simulink model "ElevatorPlant_Storage_A"  (R2015b)
(part 4 of 8)

        (junction 68772) -> (junction 68786) [order 2]
        (junction 68773) -> (junction 68779) [order 2]
        (junction 68774) -> (junction 68775) [order 2]
        (junction 68776) -> (junction 68775)
        (junction 68775) -> (junction 68777)
        (junction 68777) -> OpCl_doors.Button_detection.Max_Min_assignment.MIN [order 1] : [MIN_BUT>BUT_TEMP && not(UPDATE)]
        OpCl_doors.Button_detection.Max_Min_assignment.MIN -> (junction 68778)
        (junction 68777) -> (junction 68780) [order 2]
        (junction 68778) -> (junction 68781)
        (junction 68780) -> (junction 68779)
        (junction 68781) -> (junction 68780)
        (junction 68779) -> (junction 68782)
        (junction 68782) -> OpCl_doors.Button_detection.Max_Min_assignment.Updating_button_0 [order 1] : [MOTION==0]
        OpCl_doors.Button_detection.Max_Min_assignment.Updating_button_0 -> (junction 68783)
        (junction 68782) -> (junction 68784) [order 2]
        (junction 68783) -> (junction 68785)
        (junction 68784) -> OpCl_doors.Button_detection.Max_Min_assignment.Updating_button_1 [order 1] : [MOTION==1]
        OpCl_doors.Button_detection.Max_Min_assignment.Updating_button_1 -> (junction 68785)
        (junction 68784) -> (junction 68787) [order 2]
        (junction 68785) -> (junction 68788)
        (junction 68787) -> (junction 68786)
        (junction 68788) -> (junction 68787)
      state GoTo_PositionControl
        en:
        BUTTON=BUT_TEMP;
        FLAG=2;
      state Emergency
        en:
        FLAG_EMG=true;
        FLAG=4;
      state Timer_EME
        state Set_tmr
          en:
          Q_EME=true;
        state Counting
          en:
          ET_EME= ET_EME + 1;
          Q_EME=false;
        state Set
          en:
          IN_EME=true;
          PT_EME=3;
        (junction 68878) -> OpCl_doors.Button_detection.Timer_EME.Set_tmr [order 1] : [ET_EME==PT_EME]
        OpCl_doors.Button_detection.Timer_EME.Set_tmr -> (junction 68879)
        OpCl_doors.Button_detection.Timer_EME.Counting -> (junction 68878)
        (junction 68878) -> (junction 68879) [order 2]
        (default) -> OpCl_doors.Button_detection.Timer_EME.Set
        OpCl_doors.Button_detection.Timer_EME.Set -> (junction 68880)
        (junction 68880) -> OpCl_doors.Button_detection.Timer_EME.Counting [order 1] : [ET_EME<PT_EME]
        (junction 68880) -> (junction 68879) [order 2]
      state Not_Emergency
        en:
        IN_EME=false;
        ET_EME=0;
      state SwitchingOFF_LEDs
        en:
        LPD3=false;
        LPD2=false;
        LPS2=false;
        LPD1=false;
        LPS1=false;
        LPS0=false;
      (default) -> (junction 68479)
      (junction 68479) -> (junction 68480) [order 1] : [FLAG==1 && not(PUSHED)]
          | {BUTTON=FLOOR;
          | BUT_TEMP=BUTTON;
          | BUT_1=FLOOR;}
      (junction 68480) -> OpCl_doors.Button_detection.Timer_LL [order 1] : [not(FLAG_STOP)]
      OpCl_doors.Button_detection.Save_energy -> (junction 68481)
      OpCl_doors.Button_detection.Timer_LL -> OpCl_doors.Button_detection.Save_energy
      (junction 68480) -> (junction 68483) [order 2]
      (junction 68479) -> (junction 68482) [order 2]
      (junction 68481) -> (junction 68484)
      (junction 68483) -> (junction 68482)
      (junction 68484) -> (junction 68483)
      (junction 68482) -> OpCl_doors.Button_detection.BUTTON_CAR
      OpCl_doors.Button_detection.BUTTON_UP -> OpCl_doors.Button_detection.BUTTON_DOWN
      OpCl_doors.Button_detection.BUTTON_DOWN -> OpCl_doors.Button_detection.Max_Min_assignment
      OpCl_doors.Button_detection.Max_Min_assignment -> (junction 68485)
      OpCl_doors.Button_detection.BUTTON_CAR -> OpCl_doors.Button_detection.BUTTON_UP
      (junction 68485) -> (junction 68487)
      (junction 68487) -> (junction 68486)
      (junction 68486) -> (junction 68489)
      OpCl_doors.Button_detection.GoTo_PositionControl -> (junction 68488)
      (junction 68489) -> (junction 68490) [order 1] : [FLAG==1]
      (junction 68490) -> OpCl_doors.Button_detection.GoTo_PositionControl [order 1] : [PUSHED]
      (junction 68488) -> (junction 68492)
      (junction 68489) -> (junction 68500) [order 2]
      (junction 68490) -> (junction 68491) [order 2]
      (junction 68492) -> (junction 68491)
      (junction 68491) -> (junction 68494)
      OpCl_doors.Button_detection.Emergency -> (junction 68493)
      (junction 68494) -> OpCl_doors.Button_detection.Timer_EME [order 1] : [STOP]
          | {IN_LL=false; ET_LL=0;FLAG=1;}
      OpCl_doors.Button_detection.Timer_EME -> (junction 68495)
      (junction 68495) -> OpCl_doors.Button_detection.Emergency [order 1] : [Q_EME]
      (junction 68493) -> (junction 68497)
      (junction 68494) -> OpCl_doors.Button_detection.Not_Emergency [order 2]
      (junction 68495) -> (junction 68496) [order 2]
      (junction 68497) -> (junction 68496)
      (junction 68496) -> (junction 68499)
      OpCl_doors.Button_detection.Not_Emergency -> (junction 68499)
      OpCl_doors.Button_detection.SwitchingOFF_LEDs -> (junction 68498)
      (junction 68499) -> OpCl_doors.Button_detection.SwitchingOFF_LEDs [order 1] : [FLAG_STOP && FLAG==2]
      (junction 68498) -> (junction 68502)
      (junction 68499) -> (junction 68501) [order 2]
      (junction 68501) -> (junction 68500)
      (junction 68502) -> (junction 68501)
    state OpCl_1
      state Closing1
        state Reset
          state Reset_0
            en:
            LPS0=false;
            BUTTON_CAR(1)=false;
            BUTTON_UP(1)=false;
          state Reset_1
            en:
            LPS1=false;
            LPD1=false;
            BUTTON_CAR(2)=false;
            BUTTON_UP(2)=false;
            BUTTON_DOWN(2)=false;
          state Reset_2
            en:
            LPS2=false;
            LPD2=false;
            BUTTON_CAR(3)=false;
            BUTTON_UP(3)=false;
            BUTTON_DOWN(3)=false;
          state Reset_3
            en:
            LPD3=false;
            BUTTON_CAR(4)=false;
            BUTTON_DOWN(4)=false;
          (default) -> (junction 69446)
          (junction 69446) -> OpCl_doors.OpCl_1.Closing1.Reset.Reset_0 [order 1] : [FLOOR==0]
          OpCl_doors.OpCl_1.Closing1.Reset.Reset_0 -> (junction 69447)
          (junction 69446) -> (junction 69448) [order 2]
          (junction 69447) -> (junction 69449)
          (junction 69448) -> OpCl_doors.OpCl_1.Closing1.Reset.Reset_1 [order 1] : [FLOOR==1]
          OpCl_doors.OpCl_1.Closing1.Reset.Reset_1 -> (junction 69449)
          (junction 69448) -> (junction 69450) [order 2]
          (junction 69449) -> (junction 69451)
          (junction 69450) -> OpCl_doors.OpCl_1.Closing1.Reset.Reset_2 [order 1] : [FLOOR==2]
          OpCl_doors.OpCl_1.Closing1.Reset.Reset_2 -> (junction 69451)
          (junction 69450) -> (junction 69452) [order 2]
          (junction 69451) -> (junction 69453)
          (junction 69452) -> OpCl_doors.OpCl_1.Closing1.Reset.Reset_3 [order 1] : [FLOOR==3]
          OpCl_doors.OpCl_1.Closing1.Reset.Reset_3 -> (junction 69453)
          (junction 69452) -> (junction 69454) [order 2]
          (junction 69453) -> (junction 69455)
          (junction 69455) -> (junction 69454)
        state Timer_close
          state Set_tmr
            en: Q_cl=true;
          state Set
            en:PT_cl=5;
            IN_cl=true;
          state Counting
            en:ET_cl = ET_cl + 1;
            Q_cl=false;
          (junction 69479) -> OpCl_doors.OpCl_1.Closing1.Timer_close.Set_tmr [order 1] : [ET_cl==PT_cl]
          OpCl_doors.OpCl_1.Closing1.Timer_close.Set_tmr -> (junction 69480)
          (default) -> OpCl_doors.OpCl_1.Closing1.Timer_close.Set
          OpCl_doors.OpCl_1.Closing1.Timer_close.Counting -> (junction 69479)
          (junction 69479) -> (junction 69480) [order 2]
          OpCl_doors.OpCl_1.Closing1.Timer_close.Set -> (junction 69481)
          (junction 69481) -> OpCl_doors.OpCl_1.Closing1.Timer_close.Counting [order 1] : [ET_cl<PT_cl]
          (junction 69481) -> (junction 69480) [order 2]
        state Closing
          en: CP1=Q_cl;
        state Button_detection
          state Save_energy
            en:
            LL=not(Q_LL);
          state Timer_LL
            state Set_tmr
              en:
              Q_LL=true;
            state Counting
              en:
              ET_LL= ET_LL + 1;
              Q_LL=false;
            state Set
              en:
              IN_LL=true;
              PT_LL=10;
            (junction 69563) -> OpCl_doors.OpCl_1.Closing1.Button_detection.Timer_LL.Set_tmr [order 1] : [ET_LL==PT_LL]
            OpCl_doors.OpCl_1.Closing1.Button_detection.Timer_LL.Set_tmr -> (junction 69564)
            OpCl_doors.OpCl_1.Closing1.Button_detection.Timer_LL.Counting -> (junction 69563)
            (junction 69563) -> (junction 69564) [order 2]
            (default) -> OpCl_doors.OpCl_1.Closing1.Button_detection.Timer_LL.Set
            OpCl_doors.OpCl_1.Closing1.Button_detection.Timer_LL.Set -> (junction 69565)
            (junction 69565) -> OpCl_doors.OpCl_1.Closing1.Button_detection.Timer_LL.Counting [order 1] : [ET_LL<PT_LL]
            (junction 69565) -> (junction 69564) [order 2]
          state BUTTON_DOWN
            state Button_DOWN_1
              en:
              BUTTON_DOWN(2)=true;
              BUT_TEMP=1;
              LPD1=true;
              PUSHED=true;
              UPDATE=false;
              IN_LL=false; ET_LL=0;
            state First_but_1
              en:
              BUT_1=BUT_TEMP;
              FIRST_BUT=false;
            state Button_DOWN_2
              en:
              BUTTON_DOWN(3)=true;
              BUT_TEMP=2;
              LPD2=true;
              PUSHED=true;
              UPDATE=false;
              IN_LL=false; ET_LL=0;
            state First_but_2
              en:
              BUT_1=BUT_TEMP;
              FIRST_BUT=false;
            state Button_DOWN_3
              en:
              BUTTON_DOWN(4)=true;
              BUT_TEMP=3;
              LPD3=true;
              PUSHED=true;
              UPDATE=false;
              IN_LL=false; ET_LL=0;
            state First_but_3
              en:
              BUT_1=BUT_TEMP;
              FIRST_BUT=false;
            (default) -> (junction 69578)
            (junction 69578) -> OpCl_doors.OpCl_1.Closing1.Button_detection.BUTTON_DOWN.Button_DOWN_1 [order 1] : [PD1]
            OpCl_doors.OpCl_1.Closing1.Button_detection.BUTTON_DOWN.Button_DOWN_1 -> (junction 69579)
            (junction 69579) -> OpCl_doors.OpCl_1.Closing1.Button_detection.BUTTON_DOWN.First_but_1 [order 1] : [FIRST_BUT && not(RPC1)]
            OpCl_doors.OpCl_1.Closing1.Button_detection.BUTTON_DOWN.First_but_1 -> (junction 69580)
            (junction 69578) -> (junction 69581) [order 2]
            (junction 69579) -> (junction 69582) [order 2]
            (junction 69580) -> (junction 69583)
            (junction 69582) -> (junction 69581)
            (junction 69583) -> (junction 69582)
            (junction 69581) -> (junction 69584)
            (junction 69584) -> OpCl_doors.OpCl_1.Closing1.Button_detection.BUTTON_DOWN.Button_DOWN_2 [order 1] : [PD2]
            OpCl_doors.OpCl_1.Closing1.Button_detection.BUTTON_DOWN.Button_DOWN_2 -> (junction 69585)
            (junction 69585) -> OpCl_doors.OpCl_1.Closing1.Button_detection.BUTTON_DOWN.First_but_2 [order 1] : [FIRST_BUT && not(RPC2)]
            OpCl_doors.OpCl_1.Closing1.Button_detection.BUTTON_DOWN.First_but_2 -> (junction 69586)
            (junction 69584) -> (junction 69587) [order 2]
            (junction 69585) -> (junction 69588) [order 2]
            (junction 69586) -> (junction 69589)
            (junction 69588) -> (junction 69587)
            (junction 69589) -> (junction 69588)
            (junction 69587) -> (junction 69590)
            (junction 69590) -> OpCl_doors.OpCl_1.Closing1.Button_detection.BUTTON_DOWN.Button_DOWN_3 [order 1] : [PD3]
            OpCl_doors.OpCl_1.Closing1.Button_detection.BUTTON_DOWN.Button_DOWN_3 -> (junction 69591)
            (junction 69591) -> OpCl_doors.OpCl_1.Closing1.Button_detection.BUTTON_DOWN.First_but_3 [order 1] : [FIRST_BUT && not(RPC3)]
            OpCl_doors.OpCl_1.Closing1.Button_detection.BUTTON_DOWN.First_but_3 -> (junction 69592)
            (junction 69590) -> (junction 69593) [order 2]
            (junction 69591) -> (junction 69594) [order 2]
            (junction 69592) -> (junction 69595)
            (junction 69594) -> (junction 69593)
            (junction 69595) -> (junction 69594)
          state BUTTON_CAR
            state Button_CAR_0
              en:
              BUTTON_CAR(1)=true;
              BUT_TEMP=0;
              LPC0=true;
              PUSHED=true;
              UPDATE=false;
              IN_LL=false; ET_LL=0;
            state First_but_0
              en:
              BUT_1=BUT_TEMP;
              FIRST_BUT=false;
            state Button_CAR_1
              en:
              BUTTON_CAR(2)=true;
              BUT_TEMP=1;
              LPC1=true;
              PUSHED=true;
              UPDATE=false;
              IN_LL=false; ET_LL=0;
            state First_but_1
              en:
              BUT_1=BUT_TEMP;
              FIRST_BUT=false;
            state Button_CAR_2
              en:
              BUTTON_CAR(3)=true;
              BUT_TEMP=2;
              LPC2=true;
              PUSHED=true;
              UPDATE=false;
              IN_LL=false; ET_LL=0;
            state First_but_2
              en:
              BUT_1=BUT_TEMP;
              FIRST_BUT=false;
            state Button_CAR_3
              en:
              BUTTON_CAR(4)=true;
              BUT_TEMP=3;
              LPC3=true;
              PUSHED=true;
              UPDATE=false;
              IN_LL=false; ET_LL=0;
            state First_but_3
              en:
              BUT_1=BUT_TEMP;
              FIRST_BUT=false;
            (default) -> (junction 69633)
            (junction 69633) -> OpCl_doors.OpCl_1.Closing1.Button_detection.BUTTON_CAR.Button_CAR_0 [order 1] : [P0]
            OpCl_doors.OpCl_1.Closing1.Button_detection.BUTTON_CAR.Button_CAR_0 -> (junction 69634)
            (junction 69634) -> OpCl_doors.OpCl_1.Closing1.Button_detection.BUTTON_CAR.First_but_0 [order 1] : [FIRST_BUT && not(RPC0)]
            OpCl_doors.OpCl_1.Closing1.Button_detection.BUTTON_CAR.First_but_0 -> (junction 69635)
            (junction 69633) -> (junction 69636) [order 2]
            (junction 69634) -> (junction 69637) [order 2]
            (junction 69635) -> (junction 69638)
            (junction 69637) -> (junction 69636)
            (junction 69638) -> (junction 69637)
            (junction 69636) -> (junction 69641)
            OpCl_doors.OpCl_1.Closing1.Button_detection.BUTTON_CAR.Button_CAR_1 -> (junction 69639)
            (junction 69639) -> OpCl_doors.OpCl_1.Closing1.Button_detection.BUTTON_CAR.First_but_1 [order 1] : [FIRST_BUT && not(RPC1)]
            OpCl_doors.OpCl_1.Closing1.Button_detection.BUTTON_CAR.First_but_1 -> (junction 69640)
            (junction 69639) -> (junction 69643) [order 2]
            (junction 69640) -> (junction 69644)
            (junction 69641) -> OpCl_doors.OpCl_1.Closing1.Button_detection.BUTTON_CAR.Button_CAR_1 [order 1] : [P1]
            (junction 69641) -> (junction 69642) [order 2]
            (junction 69643) -> (junction 69642)
            (junction 69644) -> (junction 69643)
            (junction 69642) -> (junction 69645)
            (junction 69645) -> OpCl_doors.OpCl_1.Closing1.Button_detection.BUTTON_CAR.Button_CAR_2 [order 1] : [P2]
            OpCl_doors.OpCl_1.Closing1.Button_detection.BUTTON_CAR.Button_CAR_2 -> (junction 69646)
            (junction 69646) -> OpCl_doors.OpCl_1.Closing1.Button_detection.BUTTON_CAR.First_but_2 [order 1] : [FIRST_BUT && not(RPC2)]
            OpCl_doors.OpCl_1.Closing1.Button_detection.BUTTON_CAR.First_but_2 -> (junction 69647)
            (junction 69645) -> (junction 69648) [order 2]
            (junction 69646) -> (junction 69649) [order 2]
            (junction 69647) -> (junction 69650)
            (junction 69649) -> (junction 69648)
            (junction 69650) -> (junction 69649)
            (junction 69648) -> (junction 69651)
            (junction 69651) -> OpCl_doors.OpCl_1.Closing1.Button_detection.BUTTON_CAR.Button_CAR_3 [order 1] : [P3]
            OpCl_doors.OpCl_1.Closing1.Button_detection.BUTTON_CAR.Button_CAR_3 -> (junction 69652)
            (junction 69652) -> OpCl_doors.OpCl_1.Closing1.Button_detection.BUTTON_CAR.First_but_3 [order 1] : [FIRST_BUT && not(RPC3)]
            OpCl_doors.OpCl_1.Closing1.Button_detection.BUTTON_CAR.First_but_3 -> (junction 69653)
            (junction 69651) -> (junction 69654) [order 2]
            (junction 69652) -> (junction 69655) [order 2]
            (junction 69653) -> (junction 69656)
            (junction 69655) -> (junction 69654)
            (junction 69656) -> (junction 69655)
          state BUTTON_UP
            state Button_UP_0
              en:
              BUTTON_UP(1)=true;
              BUT_TEMP=0;
              LPS0=true;
              PUSHED=true;
              UPDATE=false;
              IN_LL=false; ET_LL=0;
            state First_but_0
              en:
              BUT_1=BUT_TEMP;
              FIRST_BUT=false;
            state Button_UP_1
              en:
              BUTTON_UP(2)=true;
              BUT_TEMP=1;
              LPS1=true;
              PUSHED=true;
              UPDATE=false;
              IN_LL=false; ET_LL=0;
            state First_but_1
              en:
              BUT_1=BUT_TEMP;
              FIRST_BUT=false;
            state Button_UP_2
              en:
              BUTTON_UP(3)=true;
              BUT_TEMP=2;
              LPS2=true;
              PUSHED=true;
              UPDATE=false;
              IN_LL=false; ET_LL=0;
            state First_but_2
              en:
              BUT_1=BUT_TEMP;
              FIRST_BUT=false;
            (junction 69706) -> OpCl_doors.OpCl_1.Closing1.Button_detection.BUTTON_UP.Button_UP_0 [order 1] : [PS0]
            OpCl_doors.OpCl_1.Closing1.Button_detection.BUTTON_UP.Button_UP_0 -> (junction 69707)
            (junction 69707) -> OpCl_doors.OpCl_1.Closing1.Button_detection.BUTTON_UP.First_but_0 [order 1] : [FIRST_BUT && not(RPC0)]
            OpCl_doors.OpCl_1.Closing1.Button_detection.BUTTON_UP.First_but_0 -> (junction 69708)
            (default) -> (junction 69706)
            (junction 69706) -> (junction 69711) [order 2]
            (junction 69707) -> (junction 69709) [order 2]
            (junction 69708) -> (junction 69710)
            (junction 69710) -> (junction 69709)
            (junction 69709) -> (junction 69711)
            (junction 69711) -> (junction 69712)
            (junction 69712) -> OpCl_doors.OpCl_1.Closing1.Button_detection.BUTTON_UP.Button_UP_1 [order 1] : [PS1]
            OpCl_doors.OpCl_1.Closing1.Button_detection.BUTTON_UP.Button_UP_1 -> (junction 69713)
            (junction 69713) -> OpCl_doors.OpCl_1.Closing1.Button_detection.BUTTON_UP.First_but_1 [order 1] : [FIRST_BUT && not(RPC1)]
            OpCl_doors.OpCl_1.Closing1.Button_detection.BUTTON_UP.First_but_1 -> (junction 69714)
            (junction 69712) -> (junction 69715) [order 2]
            (junction 69713) -> (junction 69716) [order 2]
            (junction 69714) -> (junction 69717)
            (junction 69716) -> (junction 69715)
            (junction 69717) -> (junction 69716)
            (junction 69715) -> (junction 69719)
            OpCl_doors.OpCl_1.Closing1.Button_detection.BUTTON_UP.First_but_2 -> (junction 69718)
            (junction 69718) -> (junction 69723)
            (junction 69719) -> OpCl_doors.OpCl_1.Closing1.Button_detection.BUTTON_UP.Button_UP_2 [order 1] : [PS2]
            OpCl_doors.OpCl_1.Closing1.Button_detection.BUTTON_UP.Button_UP_2 -> (junction 69720)
            (junction 69720) -> OpCl_doors.OpCl_1.Closing1.Button_detection.BUTTON_UP.First_but_2 [order 1] : [FIRST_BUT && not(RPC2)]
            (junction 69719) -> (junction 69721) [order 2]
            (junction 69720) -> (junction 69722) [order 2]
            (junction 69722) -> (junction 69721)
            (junction 69723) -> (junction 69722)
          state Max_Min_assignment
            state Min_but
              en:
              BUTTON=MIN_BUT;
            state Max_but
              en:
              BUTTON=MAX_BUT;
            state First_but
              en:
              BUTTON=BUT_1;
            state Max_but1
              en:
              MAX_BUT=2;
            state Max_but2
              en:
              MAX_BUT=1;
            state Max_but3
              en:
              MAX_BUT=0;
            state Min_but1
              en:
              MIN_BUT=1;
            state Min_but2
              en:
              MIN_BUT=2;
            state Min_but3
              en:
              MIN_BUT=3;
            state MAX
              en:
              MAX_BUT=BUT_TEMP;
            state MIN
              en:
              MIN_BUT=BUT_TEMP;
            state Updating_button_0
              en:
              BUTTON=MAX_BUT;
            state Updating_button_1
              en:
              BUTTON=MIN_BUT;
            (junction 69761) -> OpCl_doors.OpCl_1.Closing1.Button_detection.Max_Min_assignment.Min_but [order 1] : [(MAX_BUT-FLOOR)>(FLOOR-MIN_BUT)]
            OpCl_doors.OpCl_1.Closing1.Button_detection.Max_Min_assignment.Min_but -> (junction 69762)
            (junction 69763) -> (junction 69761) [order 1] : [not(FLAG_STOP) && MOTION==2 && FLAG==3]
            (default) -> (junction 69763)
            (junction 69761) -> (junction 69764) [order 2]
            (junction 69762) -> (junction 69765)
            (junction 69763) -> (junction 69766) [order 2]
            (junction 69764) -> OpCl_doors.OpCl_1.Closing1.Button_detection.Max_Min_assignment.Max_but [order 1] : [(MAX_BUT-FLOOR)<(FLOOR-MIN_BUT)]
            OpCl_doors.OpCl_1.Closing1.Button_detection.Max_Min_assignment.Max_but -> (junction 69765)
            (junction 69764) -> OpCl_doors.OpCl_1.Closing1.Button_detection.Max_Min_assignment.First_but [order 2]
            (junction 69765) -> (junction 69768)
            OpCl_doors.OpCl_1.Closing1.Button_detection.Max_Min_assignment.First_but -> (junction 69767)
            (junction 69767) -> (junction 69766)
            (junction 69768) -> (junction 69767)
            (junction 69766) -> (junction 69769)
            (junction 69770) -> (junction 69771) [order 1] : [MOTION==0]
                | {MOTION=1;
                | UPDATE=true;}
            (junction 69771) -> OpCl_doors.OpCl_1.Closing1.Button_detection.Max_Min_assignment.Max_but1 [order 1] : [BUTTON_UP(2)]
            OpCl_doors.OpCl_1.Closing1.Button_detection.Max_Min_assignment.Max_but1 -> (junction 69772)
            (junction 69769) -> (junction 69770) [order 1] : [BUTTON==FLOOR && EXTEND]
                | {EXTEND=false;}
            (junction 69769) -> (junction 69783) [order 2]
            (junction 69770) -> (junction 69775) [order 2]
            (junction 69771) -> (junction 69773) [order 2]
            (junction 69772) -> (junction 69774)
            (junction 69773) -> OpCl_doors.OpCl_1.Closing1.Button_detection.Max_Min_assignment.Max_but2 [order 1] : [BUTTON_UP(1)]
            OpCl_doors.OpCl_1.Closing1.Button_detection.Max_Min_assignment.Max_but2 -> (junction 69774)
            (junction 69773) -> OpCl_doors.OpCl_1.Closing1.Button_detection.Max_Min_assignment.Max_but3 [order 2]
            (junction 69774) -> (junction 69777)
            OpCl_doors.OpCl_1.Closing1.Button_detection.Max_Min_assignment.Max_but3 -> (junction 69776)
            (junction 69776) -> (junction 69775)
            (junction 69777) -> (junction 69776)
            (junction 69775) -> (junction 69778)
            (junction 69778) -> (junction 69779) [order 1] : [MOTION==1]
                | {MOTION=0;
                | UPDATE=true;}
            (junction 69779) -> OpCl_doors.OpCl_1.Closing1.Button_detection.Max_Min_assignment.Min_but1 [order 1] : [BUTTON_DOWN(1)]
            OpCl_doors.OpCl_1.Closing1.Button_detection.Max_Min_assignment.Min_but1 -> (junction 69780)
            (junction 69778) -> (junction 69784) [order 2]
            (junction 69779) -> (junction 69781) [order 2]
            (junction 69780) -> (junction 69782)
            (junction 69781) -> OpCl_doors.OpCl_1.Closing1.Button_detection.Max_Min_assignment.Min_but2 [order 1] : [BUTTON_DOWN(2)]
            OpCl_doors.OpCl_1.Closing1.Button_detection.Max_Min_assignment.Min_but2 -> (junction 69782)
            (junction 69781) -> OpCl_doors.OpCl_1.Closing1.Button_detection.Max_Min_assignment.Min_but3 [order 2]
            (junction 69782) -> (junction 69786)
            OpCl_doors.OpCl_1.Closing1.Button_detection.Max_Min_assignment.Min_but3 -> (junction 69785)
            (junction 69784) -> (junction 69783)
            (junction 69785) -> (junction 69784)
            (junction 69786) -> (junction 69785)
            (junction 69783) -> (junction 69788)
            OpCl_doors.OpCl_1.Closing1.Button_detection.Max_Min_assignment.MAX -> (junction 69787)
            (junction 69788) -> (junction 69789) [order 1] : [PUSHED]
            (junction 69789) -> (junction 69790) [order 1] : [not(BUT_TEMP==FLOOR) || not(MOTION==2)]
            (junction 69790) -> OpCl_doors.OpCl_1.Closing1.Button_detection.Max_Min_assignment.MAX [order 1] : [MAX_BUT<BUT_TEMP && not(UPDATE)]
            (junction 69787) -> (junction 69792)
            (junction 69788) -> (junction 69802) [order 2]
            (junction 69789) -> (junction 69795) [order 2]
            (junction 69790) -> (junction 69791) [order 2]
            (junction 69792) -> (junction 69791)
            (junction 69791) -> (junction 69793)
            (junction 69793) -> OpCl_doors.OpCl_1.Closing1.Button_detection.Max_Min_assignment.MIN [order 1] : [MIN_BUT>BUT_TEMP && not(UPDATE)]
            OpCl_doors.OpCl_1.Closing1.Button_detection.Max_Min_assignment.MIN -> (junction 69794)
            (junction 69793) -> (junction 69796) [order 2]
            (junction 69794) -> (junction 69797)
            (junction 69796) -> (junction 69795)
            (junction 69797) -> (junction 69796)
            (junction 69795) -> (junction 69798)
            (junction 69798) -> OpCl_doors.OpCl_1.Closing1.Button_detection.Max_Min_assignment.Updating_button_0 [order 1] : [MOTION==0]
            OpCl_doors.OpCl_1.Closing1.Button_detection.Max_Min_assignment.Updating_button_0 -> (junction 69799)
            (junction 69798) -> (junction 69800) [order 2]
            (junction 69799) -> (junction 69801)
            (junction 69800) -> OpCl_doors.OpCl_1.Closing1.Button_detection.Max_Min_assignment.Updating_button_1 [order 1] : [MOTION==1]
            OpCl_doors.OpCl_1.Closing1.Button_detection.Max_Min_assignment.Updating_button_1 -> (junction 69801)
            (junction 69800) -> (junction 69803) [order 2]
            (junction 69801) -> (junction 69804)
            (junction 69803) -> (junction 69802)
            (junction 69804) -> (junction 69803)
          state GoTo_PositionControl
            en:
            BUTTON=BUT_TEMP;
            FLAG=2;
          state Emergency
            en:
            FLAG_EMG=true;
            FLAG=4;
          state Timer_EME
            state Set_tmr
              en:
              Q_EME=true;
            state Counting
              en:
              ET_EME= ET_EME + 1;
              Q_EME=false;
            state Set
              en:
              IN_EME=true;
              PT_EME=3;
            (junction 69894) -> OpCl_doors.OpCl_1.Closing1.Button_detection.Timer_EME.Set_tmr [order 1] : [ET_EME==PT_EME]
            OpCl_doors.OpCl_1.Closing1.Button_detection.Timer_EME.Set_tmr -> (junction 69895)
            OpCl_doors.OpCl_1.Closing1.Button_detection.Timer_EME.Counting -> (junction 69894)
            (junction 69894) -> (junction 69895) [order 2]
            (default) -> OpCl_doors.OpCl_1.Closing1.Button_detection.Timer_EME.Set
            OpCl_doors.OpCl_1.Closing1.Button_detection.Timer_EME.Set -> (junction 69896)
            (junction 69896) -> OpCl_doors.OpCl_1.Closing1.Button_detection.Timer_EME.Counting [order 1] : [ET_EME<PT_EME]
            (junction 69896) -> (junction 69895) [order 2]
          state Not_Emergency
            en:
            IN_EME=false;
            ET_EME=0;
          state SwitchingOFF_LEDs
            en:
            LPD3=false;
            LPD2=false;
            LPS2=false;
            LPD1=false;
            LPS1=false;
            LPS0=false;
          (default) -> (junction 69495)
          (junction 69495) -> (junction 69496) [order 1] : [FLAG==1 && not(PUSHED)]
              | {BUTTON=FLOOR;
              | BUT_TEMP=BUTTON;
              | BUT_1=FLOOR;}
          (junction 69496) -> OpCl_doors.OpCl_1.Closing1.Button_detection.Timer_LL [order 1] : [not(FLAG_STOP)]
          OpCl_doors.OpCl_1.Closing1.Button_detection.Save_energy -> (junction 69497)
          OpCl_doors.OpCl_1.Closing1.Button_detection.Timer_LL -> OpCl_doors.OpCl_1.Closing1.Button_detection.Save_energy
          (junction 69496) -> (junction 69499) [order 2]
          (junction 69495) -> (junction 69498) [order 2]
          (junction 69497) -> (junction 69500)
          (junction 69499) -> (junction 69498)
          (junction 69500) -> (junction 69499)
          (junction 69498) -> OpCl_doors.OpCl_1.Closing1.Button_detection.BUTTON_CAR
          OpCl_doors.OpCl_1.Closing1.Button_detection.BUTTON_UP -> OpCl_doors.OpCl_1.Closing1.Button_detection.BUTTON_DOWN
          OpCl_doors.OpCl_1.Closing1.Button_detection.BUTTON_DOWN -> OpCl_doors.OpCl_1.Closing1.Button_detection.Max_Min_assignment
          OpCl_doors.OpCl_1.Closing1.Button_detection.Max_Min_assignment -> (junction 69501)
          OpCl_doors.OpCl_1.Closing1.Button_detection.BUTTON_CAR -> OpCl_doors.OpCl_1.Closing1.Button_detection.BUTTON_UP
          (junction 69501) -> (junction 69503)
          (junction 69503) -> (junction 69502)
          (junction 69502) -> (junction 69505)
          OpCl_doors.OpCl_1.Closing1.Button_detection.GoTo_PositionControl -> (junction 69504)
          (junction 69505) -> (junction 69506) [order 1] : [FLAG==1]
          (junction 69506) -> OpCl_doors.OpCl_1.Closing1.Button_detection.GoTo_PositionControl [order 1] : [PUSHED]
          (junction 69504) -> (junction 69508)
          (junction 69505) -> (junction 69516) [order 2]
          (junction 69506) -> (junction 69507) [order 2]
          (junction 69508) -> (junction 69507)
          (junction 69507) -> (junction 69510)
          OpCl_doors.OpCl_1.Closing1.Button_detection.Emergency -> (junction 69509)
          (junction 69510) -> OpCl_doors.OpCl_1.Closing1.Button_detection.Timer_EME [order 1] : [STOP]
              | {IN_LL=false; ET_LL=0;FLAG=1;}
          OpCl_doors.OpCl_1.Closing1.Button_detection.Timer_EME -> (junction 69511)
          (junction 69511) -> OpCl_doors.OpCl_1.Closing1.Button_detection.Emergency [order 1] : [Q_EME]
          (junction 69509) -> (junction 69513)
          (junction 69510) -> OpCl_doors.OpCl_1.Closing1.Button_detection.Not_Emergency [order 2]
          (junction 69511) -> (junction 69512) [order 2]
          (junction 69513) -> (junction 69512)
          (junction 69512) -> (junction 69515)
          OpCl_doors.OpCl_1.Closing1.Button_detection.Not_Emergency -> (junction 69515)
          OpCl_doors.OpCl_1.Closing1.Button_detection.SwitchingOFF_LEDs -> (junction 69514)
          (junction 69515) -> OpCl_doors.OpCl_1.Closing1.Button_detection.SwitchingOFF_LEDs [order 1] : [FLAG_STOP && FLAG==2]
          (junction 69514) -> (junction 69518)
          (junction 69515) -> (junction 69517) [order 2]
          (junction 69517) -> (junction 69516)
          (junction 69518) -> (junction 69517)
        state Extending
          en:
          EXTEND=true;
        state Stop_Closing
          en:
          CP1=false;
          FLAG_OD=false;
          OBS=false;
          ET_cl=0;
          IN_cl=false;
        state GoTo_PositionControl
          en: FLAG=2;
        state GoTo_BUttonDetection
          en:
          MOTION=2;
          MAX_BUT=0;
          MIN_BUT=3;
          PUSHED=false;
          FIRST_BUT=true;
          FLAG=1;
          UPDATE=false;
        state Closing1
          en:CP1=true;
        state Stop_Closing1
          en:CP1=false;
        OpCl_doors.OpCl_1.Closing1.Reset -> OpCl_doors.OpCl_1.Closing1.Timer_close
        (default) -> (junction 69406)
        (junction 69406) -> OpCl_doors.OpCl_1.Closing1.Reset [order 1] : [not(FLAG==0) && not(FLAG==4)]
        OpCl_doors.OpCl_1.Closing1.Timer_close -> (junction 69407)
        (junction 69407) -> OpCl_doors.OpCl_1.Closing1.Closing [order 1] : [not(PC1)]
        OpCl_doors.OpCl_1.Closing1.Button_detection -> (junction 69408)
        OpCl_doors.OpCl_1.Closing1.Closing -> OpCl_doors.OpCl_1.Closing1.Button_detection
        (junction 69406) -> (junction 69416) [order 2]
        (junction 69407) -> (junction 69409) [order 2]
        (junction 69408) -> (junction 69414)
        (junction 69409) -> OpCl_doors.OpCl_1.Closing1.Extending [order 1] : [BUTTON==FLOOR]
        (junction 69409) -> (junction 69411) [order 2]
        OpCl_doors.OpCl_1.Closing1.Extending -> (junction 69410)
        (junction 69410) -> (junction 69411)
        (junction 69411) -> OpCl_doors.OpCl_1.Closing1.Stop_Closing
        OpCl_doors.OpCl_1.Closing1.Stop_Closing -> (junction 69412)
        (junction 69412) -> OpCl_doors.OpCl_1.Closing1.GoTo_PositionControl [order 2]
        (junction 69412) -> OpCl_doors.OpCl_1.Closing1.GoTo_BUttonDetection [order 1] : [not(BUTTON_CAR(1) || BUTTON_CAR(2) || BUTTON_CAR(3) || BUTTON_CAR(4) || BUTTON_UP(1) || BUTTON_UP(2) || BUTTON_UP(3) || BUTTON_DOWN(2) || BUTTON_DOWN(3) || BUTTON_DOWN(4))]
        OpCl_doors.OpCl_1.Closing1.GoTo_PositionControl -> (junction 69413)
        OpCl_doors.OpCl_1.Closing1.GoTo_BUttonDetection -> (junction 69413)
        (junction 69413) -> (junction 69414)
        (junction 69414) -> (junction 69415)
        (junction 69415) -> (junction 69417)
        (junction 69416) -> OpCl_doors.OpCl_1.Closing1.Closing1 [order 1] : [not(PC1)]
        OpCl_doors.OpCl_1.Closing1.Closing1 -> (junction 69417)
        (junction 69416) -> OpCl_doors.OpCl_1.Closing1.Stop_Closing1 [order 2]
        OpCl_doors.OpCl_1.Closing1.Stop_Closing1 -> (junction 69417)
      state StopClosing
        en: CP1=false;
        FLAG_OD=false;
      state Opening1
        state Opening
          en:AP1=Q_op;
        state People_IN
          state Check_People_IN
            en:
            COUNTER_IN=false;
          state People_KID_IN
            en:
            WEIGHT=WEIGHT+30;
            KIDS=KIDS+1;
          state People_WOMAN_IN
            en:
            WEIGHT=WEIGHT+55;
            WOMEN=WOMEN+1;
          state People_MAN_IN
            en:
            WEIGHT=WEIGHT+75;
            MEN=MEN+1;
          state People_FATGUY_IN
            en:
            WEIGHT=WEIGHT+100;
            FATGUYS=FATGUYS+1;
          state Re_Ready_IN
            en:
            COUNTER_IN=true;
          (default) -> (junction 88272)
          (junction 88272) -> OpCl_doors.OpCl_1.Opening1.People_IN.Check_People_IN [order 1] : [COUNTER_IN]
          OpCl_doors.OpCl_1.Opening1.People_IN.Check_People_IN -> (junction 88273)
          (junction 88273) -> OpCl_doors.OpCl_1.Opening1.People_IN.People_KID_IN [order 1] : [KID_IN]
          OpCl_doors.OpCl_1.Opening1.People_IN.People_KID_IN -> (junction 88274)
          (junction 88272) -> (junction 88281) [order 2]
          (junction 88273) -> (junction 88275) [order 2]
          (junction 88274) -> (junction 88276)
          (junction 88275) -> OpCl_doors.OpCl_1.Opening1.People_IN.People_WOMAN_IN [order 1] : [WOMAN_IN]
          OpCl_doors.OpCl_1.Opening1.People_IN.People_WOMAN_IN -> (junction 88276)
          (junction 88275) -> (junction 88277) [order 2]
          (junction 88276) -> (junction 88278)
          (junction 88277) -> OpCl_doors.OpCl_1.Opening1.People_IN.People_MAN_IN [order 1] : [MAN_IN]
          OpCl_doors.OpCl_1.Opening1.People_IN.People_MAN_IN -> (junction 88278)
          (junction 88277) -> (junction 88279) [order 2]
          (junction 88278) -> (junction 88280)
          (junction 88279) -> OpCl_doors.OpCl_1.Opening1.People_IN.People_FATGUY_IN [order 1] : [FATGUY_IN]
          OpCl_doors.OpCl_1.Opening1.People_IN.People_FATGUY_IN -> (junction 88280)
          (junction 88279) -> (junction 88282) [order 2]
          (junction 88280) -> (junction 88283)
          (junction 88282) -> (junction 88281)
          (junction 88283) -> (junction 88282)
          (junction 88281) -> (junction 88284)
          (junction 88284) -> OpCl_doors.OpCl_1.Opening1.People_IN.Re_Ready_IN [order 1] : [not(KID_IN|| WOMAN_IN || MAN_IN || FATGUY_IN)]
          (junction 88284) -> (junction 88285) [order 2]
          OpCl_doors.OpCl_1.Opening1.People_IN.Re_Ready_IN -> (junction 88286)
          (junction 88286) -> (junction 88285)
        state Timer_open
          state Set_tmr
            en: Q_op=true;
          state Set
            en:PT_op=2;
            IN_op=true;
          state Counting
            en:ET_op = ET_op + 1;
            Q_op=false;
          (junction 88321) -> OpCl_doors.OpCl_1.Opening1.Timer_open.Set_tmr [order 1] : [ET_op==PT_op]
          OpCl_doors.OpCl_1.Opening1.Timer_open.Set_tmr -> (junction 88322)
          (default) -> OpCl_doors.OpCl_1.Opening1.Timer_open.Set
          OpCl_doors.OpCl_1.Opening1.Timer_open.Counting -> (junction 88321)
          (junction 88321) -> (junction 88322) [order 2]
          OpCl_doors.OpCl_1.Opening1.Timer_open.Set -> (junction 88323)
          (junction 88323) -> OpCl_doors.OpCl_1.Opening1.Timer_open.Counting [order 1] : [ET_op<PT_op]
          (junction 88323) -> (junction 88322) [order 2]
        state Stop_Opening
          en:AP1=false;
          FLAG_OD=true;
          OBS=true;
          IN_op=false;
          ET_op=0;
        state People_OUT
          state Check_People_OUT
            en:
            COUNTER_OUT=false;
          state People_KID_OUT
            en:
            WEIGHT=WEIGHT-30;
            KIDS=KIDS-1;
          state People_WOMAN_OUT
            en:
            WEIGHT=WEIGHT-55;
            WOMEN=WOMEN-1;
          state People_MAN_OUT
            en:
            WEIGHT=WEIGHT-75;
            MEN=MEN-1;
          state People_FATGUY_OUT
            en:
            WEIGHT=WEIGHT-100;
            FATGUYS=FATGUYS-1;
          state Re_Ready_OUT
            en:
            COUNTER_OUT=true;
          (default) -> (junction 88337)
          (junction 88337) -> OpCl_doors.OpCl_1.Opening1.People_OUT.Check_People_OUT [order 1] : [COUNTER_OUT]
          OpCl_doors.OpCl_1.Opening1.People_OUT.Check_People_OUT -> (junction 88338)
          (junction 88338) -> OpCl_doors.OpCl_1.Opening1.People_OUT.People_KID_OUT [order 1] : [KID_OUT && KIDS>0 ]
          OpCl_doors.OpCl_1.Opening1.People_OUT.People_KID_OUT -> (junction 88339)
          (junction 88337) -> (junction 88346) [order 2]
          (junction 88338) -> (junction 88340) [order 2]
          (junction 88339) -> (junction 88341)
          (junction 88340) -> OpCl_doors.OpCl_1.Opening1.People_OUT.People_WOMAN_OUT [order 1] : [WOMAN_OUT && WOMEN>0]
          OpCl_doors.OpCl_1.Opening1.People_OUT.People_WOMAN_OUT -> (junction 88341)
          (junction 88341) -> (junction 88343)
          (junction 88340) -> (junction 88342) [order 2]
          (junction 88342) -> OpCl_doors.OpCl_1.Opening1.People_OUT.People_MAN_OUT [order 1] : [MAN_OUT && MEN>0]
          OpCl_doors.OpCl_1.Opening1.People_OUT.People_MAN_OUT -> (junction 88343)
          (junction 88342) -> (junction 88344) [order 2]
          (junction 88343) -> (junction 88345)
          (junction 88344) -> OpCl_doors.OpCl_1.Opening1.People_OUT.People_FATGUY_OUT [order 1] : [FATGUY_OUT && FATGUYS>0]
          OpCl_doors.OpCl_1.Opening1.People_OUT.People_FATGUY_OUT -> (junction 88345)
          (junction 88344) -> (junction 88347) [order 2]
          (junction 88345) -> (junction 88348)
          (junction 88347) -> (junction 88346)
          (junction 88348) -> (junction 88347)
          (junction 88346) -> (junction 88349)
          (junction 88349) -> OpCl_doors.OpCl_1.Opening1.People_OUT.Re_Ready_OUT [order 1] : [not(KID_OUT || WOMAN_OUT || MAN_OUT || FATGUY_OUT)]
          (junction 88349) -> (junction 88350) [order 2]
          OpCl_doors.OpCl_1.Opening1.People_OUT.Re_Ready_OUT -> (junction 88351)
          (junction 88351) -> (junction 88350)
        state Button_detection
          state Save_energy
            en:
            LL=not(Q_LL);
          state Timer_LL
            state Set_tmr
              en:
              Q_LL=true;
            state Counting
              en:
              ET_LL= ET_LL + 1;
              Q_LL=false;
            state Set
              en:
              IN_LL=true;
              PT_LL=10;
            (junction 88454) -> OpCl_doors.OpCl_1.Opening1.Button_detection.Timer_LL.Set_tmr [order 1] : [ET_LL==PT_LL]
            OpCl_doors.OpCl_1.Opening1.Button_detection.Timer_LL.Set_tmr -> (junction 88455)
            OpCl_doors.OpCl_1.Opening1.Button_detection.Timer_LL.Counting -> (junction 88454)
            (junction 88454) -> (junction 88455) [order 2]
            (default) -> OpCl_doors.OpCl_1.Opening1.Button_detection.Timer_LL.Set
            OpCl_doors.OpCl_1.Opening1.Button_detection.Timer_LL.Set -> (junction 88456)
            (junction 88456) -> OpCl_doors.OpCl_1.Opening1.Button_detection.Timer_LL.Counting [order 1] : [ET_LL<PT_LL]
            (junction 88456) -> (junction 88455) [order 2]
          state BUTTON_DOWN
            state Button_DOWN_1
              en:
              BUTTON_DOWN(2)=true;
              BUT_TEMP=1;
              LPD1=true;
              PUSHED=true;
              UPDATE=false;
              IN_LL=false; ET_LL=0;
            state First_but_1
              en:
              BUT_1=BUT_TEMP;
              FIRST_BUT=false;
            state Button_DOWN_2
              en:
              BUTTON_DOWN(3)=true;
              BUT_TEMP=2;
              LPD2=true;
              PUSHED=true;
              UPDATE=false;
              IN_LL=false; ET_LL=0;
            state First_but_2
              en:
              BUT_1=BUT_TEMP;
              FIRST_BUT=false;
            state Button_DOWN_3
              en:
              BUTTON_DOWN(4)=true;
              BUT_TEMP=3;
              LPD3=true;
              PUSHED=true;
              UPDATE=false;
              IN_LL=false; ET_LL=0;
            state First_but_3
              en:
              BUT_1=BUT_TEMP;
              FIRST_BUT=false;
            (default) -> (junction 88469)
            (junction 88469) -> OpCl_doors.OpCl_1.Opening1.Button_detection.BUTTON_DOWN.Button_DOWN_1 [order 1] : [PD1]
            OpCl_doors.OpCl_1.Opening1.Button_detection.BUTTON_DOWN.Button_DOWN_1 -> (junction 88470)
            (junction 88470) -> OpCl_doors.OpCl_1.Opening1.Button_detection.BUTTON_DOWN.First_but_1 [order 1] : [FIRST_BUT && not(RPC1)]
            OpCl_doors.OpCl_1.Opening1.Button_detection.BUTTON_DOWN.First_but_1 -> (junction 88471)
            (junction 88469) -> (junction 88472) [order 2]
            (junction 88470) -> (junction 88473) [order 2]
            (junction 88471) -> (junction 88474)
            (junction 88473) -> (junction 88472)
            (junction 88474) -> (junction 88473)
            (junction 88472) -> (junction 88475)
            (junction 88475) -> OpCl_doors.OpCl_1.Opening1.Button_detection.BUTTON_DOWN.Button_DOWN_2 [order 1] : [PD2]
            OpCl_doors.OpCl_1.Opening1.Button_detection.BUTTON_DOWN.Button_DOWN_2 -> (junction 88476)
            (junction 88476) -> OpCl_doors.OpCl_1.Opening1.Button_detection.BUTTON_DOWN.First_but_2 [order 1] : [FIRST_BUT && not(RPC2)]
            OpCl_doors.OpCl_1.Opening1.Button_detection.BUTTON_DOWN.First_but_2 -> (junction 88477)
            (junction 88475) -> (junction 88478) [order 2]
            (junction 88476) -> (junction 88479) [order 2]
            (junction 88477) -> (junction 88480)
            (junction 88479) -> (junction 88478)
            (junction 88480) -> (junction 88479)
            (junction 88478) -> (junction 88481)
            (junction 88481) -> OpCl_doors.OpCl_1.Opening1.Button_detection.BUTTON_DOWN.Button_DOWN_3 [order 1] : [PD3]
            OpCl_doors.OpCl_1.Opening1.Button_detection.BUTTON_DOWN.Button_DOWN_3 -> (junction 88482)
            (junction 88482) -> OpCl_doors.OpCl_1.Opening1.Button_detection.BUTTON_DOWN.First_but_3 [order 1] : [FIRST_BUT && not(RPC3)]
            OpCl_doors.OpCl_1.Opening1.Button_detection.BUTTON_DOWN.First_but_3 -> (junction 88483)
            (junction 88481) -> (junction 88484) [order 2]
            (junction 88482) -> (junction 88485) [order 2]
            (junction 88483) -> (junction 88486)
            (junction 88485) -> (junction 88484)
            (junction 88486) -> (junction 88485)
          state BUTTON_CAR
            state Button_CAR_0
              en:
              BUTTON_CAR(1)=true;
              BUT_TEMP=0;
              LPC0=true;
              PUSHED=true;
              UPDATE=false;
              IN_LL=false; ET_LL=0;
            state First_but_0
              en:
              BUT_1=BUT_TEMP;
              FIRST_BUT=false;
            state Button_CAR_1
              en:
              BUTTON_CAR(2)=true;
              BUT_TEMP=1;
              LPC1=true;
              PUSHED=true;
              UPDATE=false;
              IN_LL=false; ET_LL=0;
            state First_but_1
              en:
              BUT_1=BUT_TEMP;
              FIRST_BUT=false;
            state Button_CAR_2
              en:
              BUTTON_CAR(3)=true;
              BUT_TEMP=2;
              LPC2=true;
              PUSHED=true;
              UPDATE=false;
              IN_LL=false; ET_LL=0;
            state First_but_2
              en:
              BUT_1=BUT_TEMP;
              FIRST_BUT=false;
            state Button_CAR_3
              en:
              BUTTON_CAR(4)=true;
              BUT_TEMP=3;
              LPC3=true;
              PUSHED=true;
              UPDATE=false;
              IN_LL=false; ET_LL=0;
            state First_but_3
              en:
              BUT_1=BUT_TEMP;
              FIRST_BUT=false;
            (default) -> (junction 88524)
            (junction 88524) -> OpCl_doors.OpCl_1.Opening1.Button_detection.BUTTON_CAR.Button_CAR_0 [order 1] : [P0]
            OpCl_doors.OpCl_1.Opening1.Button_detection.BUTTON_CAR.Button_CAR_0 -> (junction 88525)
            (junction 88525) -> OpCl_doors.OpCl_1.Opening1.Button_detection.BUTTON_CAR.First_but_0 [order 1] : [FIRST_BUT && not(RPC0)]
            OpCl_doors.OpCl_1.Opening1.Button_detection.BUTTON_CAR.First_but_0 -> (junction 88526)
            (junction 88524) -> (junction 88527) [order 2]
            (junction 88525) -> (junction 88528) [order 2]
            (junction 88526) -> (junction 88529)
            (junction 88528) -> (junction 88527)
            (junction 88529) -> (junction 88528)
            (junction 88527) -> (junction 88532)
            OpCl_doors.OpCl_1.Opening1.Button_detection.BUTTON_CAR.Button_CAR_1 -> (junction 88530)
            (junction 88530) -> OpCl_doors.OpCl_1.Opening1.Button_detection.BUTTON_CAR.First_but_1 [order 1] : [FIRST_BUT && not(RPC1)]
            OpCl_doors.OpCl_1.Opening1.Button_detection.BUTTON_CAR.First_but_1 -> (junction 88531)
            (junction 88530) -> (junction 88534) [order 2]
            (junction 88531) -> (junction 88535)
            (junction 88532) -> OpCl_doors.OpCl_1.Opening1.Button_detection.BUTTON_CAR.Button_CAR_1 [order 1] : [P1]
            (junction 88532) -> (junction 88533) [order 2]
            (junction 88534) -> (junction 88533)
            (junction 88535) -> (junction 88534)
            (junction 88533) -> (junction 88536)
            (junction 88536) -> OpCl_doors.OpCl_1.Opening1.Button_detection.BUTTON_CAR.Button_CAR_2 [order 1] : [P2]
            OpCl_doors.OpCl_1.Opening1.Button_detection.BUTTON_CAR.Button_CAR_2 -> (junction 88537)
            (junction 88537) -> OpCl_doors.OpCl_1.Opening1.Button_detection.BUTTON_CAR.First_but_2 [order 1] : [FIRST_BUT && not(RPC2)]
            OpCl_doors.OpCl_1.Opening1.Button_detection.BUTTON_CAR.First_but_2 -> (junction 88538)
            (junction 88536) -> (junction 88539) [order 2]
            (junction 88537) -> (junction 88540) [order 2]
            (junction 88538) -> (junction 88541)
            (junction 88540) -> (junction 88539)
            (junction 88541) -> (junction 88540)
            (junction 88539) -> (junction 88542)
            (junction 88542) -> OpCl_doors.OpCl_1.Opening1.Button_detection.BUTTON_CAR.Button_CAR_3 [order 1] : [P3]
            OpCl_doors.OpCl_1.Opening1.Button_detection.BUTTON_CAR.Button_CAR_3 -> (junction 88543)
            (junction 88543) -> OpCl_doors.OpCl_1.Opening1.Button_detection.BUTTON_CAR.First_but_3 [order 1] : [FIRST_BUT && not(RPC3)]
            OpCl_doors.OpCl_1.Opening1.Button_detection.BUTTON_CAR.First_but_3 -> (junction 88544)
            (junction 88542) -> (junction 88545) [order 2]
            (junction 88543) -> (junction 88546) [order 2]
            (junction 88544) -> (junction 88547)
            (junction 88546) -> (junction 88545)
            (junction 88547) -> (junction 88546)
          state BUTTON_UP
            state Button_UP_0
              en:
              BUTTON_UP(1)=true;
              BUT_TEMP=0;
              LPS0=true;
              PUSHED=true;
              UPDATE=false;
              IN_LL=false; ET_LL=0;
            state First_but_0
              en:
              BUT_1=BUT_TEMP;
              FIRST_BUT=false;
            state Button_UP_1
              en:
              BUTTON_UP(2)=true;
              BUT_TEMP=1;
              LPS1=true;
              PUSHED=true;
              UPDATE=false;
              IN_LL=false; ET_LL=0;
            state First_but_1
              en:
              BUT_1=BUT_TEMP;
              FIRST_BUT=false;
            state Button_UP_2
              en:
              BUTTON_UP(3)=true;
              BUT_TEMP=2;
              LPS2=true;
              PUSHED=true;
              UPDATE=false;
              IN_LL=false; ET_LL=0;
            state First_but_2
              en:
              BUT_1=BUT_TEMP;
              FIRST_BUT=false;
            (junction 88597) -> OpCl_doors.OpCl_1.Opening1.Button_detection.BUTTON_UP.Button_UP_0 [order 1] : [PS0]
            OpCl_doors.OpCl_1.Opening1.Button_detection.BUTTON_UP.Button_UP_0 -> (junction 88598)
            (junction 88598) -> OpCl_doors.OpCl_1.Opening1.Button_detection.BUTTON_UP.First_but_0 [order 1] : [FIRST_BUT && not(RPC0)]
            OpCl_doors.OpCl_1.Opening1.Button_detection.BUTTON_UP.First_but_0 -> (junction 88599)
            (default) -> (junction 88597)
            (junction 88597) -> (junction 88602) [order 2]
            (junction 88598) -> (junction 88600) [order 2]
            (junction 88599) -> (junction 88601)
            (junction 88601) -> (junction 88600)
            (junction 88600) -> (junction 88602)
            (junction 88602) -> (junction 88603)
            (junction 88603) -> OpCl_doors.OpCl_1.Opening1.Button_detection.BUTTON_UP.Button_UP_1 [order 1] : [PS1]
            OpCl_doors.OpCl_1.Opening1.Button_detection.BUTTON_UP.Button_UP_1 -> (junction 88604)
            (junction 88604) -> OpCl_doors.OpCl_1.Opening1.Button_detection.BUTTON_UP.First_but_1 [order 1] : [FIRST_BUT && not(RPC1)]
            OpCl_doors.OpCl_1.Opening1.Button_detection.BUTTON_UP.First_but_1 -> (junction 88605)
            (junction 88603) -> (junction 88606) [order 2]
            (junction 88604) -> (junction 88607) [order 2]
            (junction 88605) -> (junction 88608)
            (junction 88607) -> (junction 88606)
            (junction 88608) -> (junction 88607)
            (junction 88606) -> (junction 88610)
            OpCl_doors.OpCl_1.Opening1.Button_detection.BUTTON_UP.First_but_2 -> (junction 88609)
            (junction 88609) -> (junction 88614)
            (junction 88610) -> OpCl_doors.OpCl_1.Opening1.Button_detection.BUTTON_UP.Button_UP_2 [order 1] : [PS2]
            OpCl_doors.OpCl_1.Opening1.Button_detection.BUTTON_UP.Button_UP_2 -> (junction 88611)
            (junction 88611) -> OpCl_doors.OpCl_1.Opening1.Button_detection.BUTTON_UP.First_but_2 [order 1] : [FIRST_BUT && not(RPC2)]
            (junction 88610) -> (junction 88612) [order 2]
            (junction 88611) -> (junction 88613) [order 2]
            (junction 88613) -> (junction 88612)
            (junction 88614) -> (junction 88613)
          state Max_Min_assignment
            state Min_but
              en:
              BUTTON=MIN_BUT;
            state Max_but
              en:
              BUTTON=MAX_BUT;
            state First_but
              en:
              BUTTON=BUT_1;
            state Max_but1
              en:
              MAX_BUT=2;
            state Max_but2
              en:
              MAX_BUT=1;
            state Max_but3
              en:
              MAX_BUT=0;
            state Min_but1
              en:
              MIN_BUT=1;
            state Min_but2
              en:
              MIN_BUT=2;
            state Min_but3
              en:
              MIN_BUT=3;
            state MAX
              en:
              MAX_BUT=BUT_TEMP;
            state MIN
              en:
              MIN_BUT=BUT_TEMP;
            state Updating_button_0
              en:
              BUTTON=MAX_BUT;
            state Updating_button_1
              en:
              BUTTON=MIN_BUT;
            (junction 88652) -> OpCl_doors.OpCl_1.Opening1.Button_detection.Max_Min_assignment.Min_but [order 1] : [(MAX_BUT-FLOOR)>(FLOOR-MIN_BUT)]
            OpCl_doors.OpCl_1.Opening1.Button_detection.Max_Min_assignment.Min_but -> (junction 88653)
            (junction 88654) -> (junction 88652) [order 1] : [not(FLAG_STOP) && MOTION==2 && FLAG==3]
            (default) -> (junction 88654)
            (junction 88652) -> (junction 88655) [order 2]
            (junction 88653) -> (junction 88656)
            (junction 88654) -> (junction 88657) [order 2]
            (junction 88655) -> OpCl_doors.OpCl_1.Opening1.Button_detection.Max_Min_assignment.Max_but [order 1] : [(MAX_BUT-FLOOR)<(FLOOR-MIN_BUT)]
            OpCl_doors.OpCl_1.Opening1.Button_detection.Max_Min_assignment.Max_but -> (junction 88656)
            (junction 88655) -> OpCl_doors.OpCl_1.Opening1.Button_detection.Max_Min_assignment.First_but [order 2]
            (junction 88656) -> (junction 88659)
            OpCl_doors.OpCl_1.Opening1.Button_detection.Max_Min_assignment.First_but -> (junction 88658)
            (junction 88658) -> (junction 88657)
            (junction 88659) -> (junction 88658)
            (junction 88657) -> (junction 88660)
            (junction 88661) -> (junction 88662) [order 1] : [MOTION==0]
                | {MOTION=1;
                | UPDATE=true;}
            (junction 88662) -> OpCl_doors.OpCl_1.Opening1.Button_detection.Max_Min_assignment.Max_but1 [order 1] : [BUTTON_UP(2)]
            OpCl_doors.OpCl_1.Opening1.Button_detection.Max_Min_assignment.Max_but1 -> (junction 88663)
            (junction 88660) -> (junction 88661) [order 1] : [BUTTON==FLOOR && EXTEND]
                | {EXTEND=false;}
            (junction 88660) -> (junction 88674) [order 2]
            (junction 88661) -> (junction 88666) [order 2]
            (junction 88662) -> (junction 88664) [order 2]
            (junction 88663) -> (junction 88665)
            (junction 88664) -> OpCl_doors.OpCl_1.Opening1.Button_detection.Max_Min_assignment.Max_but2 [order 1] : [BUTTON_UP(1)]
            OpCl_doors.OpCl_1.Opening1.Button_detection.Max_Min_assignment.Max_but2 -> (junction 88665)
            (junction 88664) -> OpCl_doors.OpCl_1.Opening1.Button_detection.Max_Min_assignment.Max_but3 [order 2]
            (junction 88665) -> (junction 88668)
            OpCl_doors.OpCl_1.Opening1.Button_detection.Max_Min_assignment.Max_but3 -> (junction 88667)
            (junction 88667) -> (junction 88666)
            (junction 88668) -> (junction 88667)
            (junction 88666) -> (junction 88669)
            (junction 88669) -> (junction 88670) [order 1] : [MOTION==1]
                | {MOTION=0;
                | UPDATE=true;}
            (junction 88670) -> OpCl_doors.OpCl_1.Opening1.Button_detection.Max_Min_assignment.Min_but1 [order 1] : [BUTTON_DOWN(1)]
            OpCl_doors.OpCl_1.Opening1.Button_detection.Max_Min_assignment.Min_but1 -> (junction 88671)
            (junction 88669) -> (junction 88675) [order 2]
            (junction 88670) -> (junction 88672) [order 2]
            (junction 88671) -> (junction 88673)
            (junction 88672) -> OpCl_doors.OpCl_1.Opening1.Button_detection.Max_Min_assignment.Min_but2 [order 1] : [BUTTON_DOWN(2)]
            OpCl_doors.OpCl_1.Opening1.Button_detection.Max_Min_assignment.Min_but2 -> (junction 88673)
            (junction 88672) -> OpCl_doors.OpCl_1.Opening1.Button_detection.Max_Min_assignment.Min_but3 [order 2]
            (junction 88673) -> (junction 88677)
            OpCl_doors.OpCl_1.Opening1.Button_detection.Max_Min_assignment.Min_but3 -> (junction 88676)
            (junction 88675) -> (junction 88674)
            (junction 88676) -> (junction 88675)
            (junction 88677) -> (junction 88676)
            (junction 88674) -> (junction 88679)
            OpCl_doors.OpCl_1.Opening1.Button_detection.Max_Min_assignment.MAX -> (junction 88678)
            (junction 88679) -> (junction 88680) [order 1] : [PUSHED]
            (junction 88680) -> (junction 88681) [order 1] : [not(BUT_TEMP==FLOOR) || not(MOTION==2)]
            (junction 88681) -> OpCl_doors.OpCl_1.Opening1.Button_detection.Max_Min_assignment.MAX [order 1] : [MAX_BUT<BUT_TEMP && not(UPDATE)]
            (junction 88678) -> (junction 88683)
            (junction 88679) -> (junction 88693) [order 2]
            (junction 88680) -> (junction 88686) [order 2]
            (junction 88681) -> (junction 88682) [order 2]
            (junction 88683) -> (junction 88682)
            (junction 88682) -> (junction 88684)
            (junction 88684) -> OpCl_doors.OpCl_1.Opening1.Button_detection.Max_Min_assignment.MIN [order 1] : [MIN_BUT>BUT_TEMP && not(UPDATE)]
            OpCl_doors.OpCl_1.Opening1.Button_detection.Max_Min_assignment.MIN -> (junction 88685)
            (junction 88684) -> (junction 88687) [order 2]
            (junction 88685) -> (junction 88688)
            (junction 88687) -> (junction 88686)
            (junction 88688) -> (junction 88687)
            (junction 88686) -> (junction 88689)
            (junction 88689) -> OpCl_doors.OpCl_1.Opening1.Button_detection.Max_Min_assignment.Updating_button_0 [order 1] : [MOTION==0]
            OpCl_doors.OpCl_1.Opening1.Button_detection.Max_Min_assignment.Updating_button_0 -> (junction 88690)
            (junction 88689) -> (junction 88691) [order 2]
            (junction 88690) -> (junction 88692)
            (junction 88691) -> OpCl_doors.OpCl_1.Opening1.Button_detection.Max_Min_assignment.Updating_button_1 [order 1] : [MOTION==1]
            OpCl_doors.OpCl_1.Opening1.Button_detection.Max_Min_assignment.Updating_button_1 -> (junction 88692)
            (junction 88691) -> (junction 88694) [order 2]
            (junction 88692) -> (junction 88695)
            (junction 88694) -> (junction 88693)
            (junction 88695) -> (junction 88694)
          state GoTo_PositionControl
            en:
            BUTTON=BUT_TEMP;
            FLAG=2;
          state Emergency
            en:
            FLAG_EMG=true;
            FLAG=4;
          state Timer_EME
            state Set_tmr
              en:
              Q_EME=true;
            state Counting
              en:
              ET_EME= ET_EME + 1;
              Q_EME=false;
            state Set
              en:
              IN_EME=true;
              PT_EME=3;
            (junction 88785) -> OpCl_doors.OpCl_1.Opening1.Button_detection.Timer_EME.Set_tmr [order 1] : [ET_EME==PT_EME]
            OpCl_doors.OpCl_1.Opening1.Button_detection.Timer_EME.Set_tmr -> (junction 88786)
            OpCl_doors.OpCl_1.Opening1.Button_detection.Timer_EME.Counting -> (junction 88785)
            (junction 88785) -> (junction 88786) [order 2]
            (default) -> OpCl_doors.OpCl_1.Opening1.Button_detection.Timer_EME.Set
            OpCl_doors.OpCl_1.Opening1.Button_detection.Timer_EME.Set -> (junction 88787)
            (junction 88787) -> OpCl_doors.OpCl_1.Opening1.Button_detection.Timer_EME.Counting [order 1] : [ET_EME<PT_EME]
            (junction 88787) -> (junction 88786) [order 2]
          state Not_Emergency
            en:
            IN_EME=false;
            ET_EME=0;
          state SwitchingOFF_LEDs
            en:
            LPD3=false;
            LPD2=false;
            LPS2=false;
            LPD1=false;
            LPS1=false;
            LPS0=false;
          (default) -> (junction 88386)
          (junction 88386) -> (junction 88387) [order 1] : [FLAG==1 && not(PUSHED)]
              | {BUTTON=FLOOR;
              | BUT_TEMP=BUTTON;
              | BUT_1=FLOOR;}
          (junction 88387) -> OpCl_doors.OpCl_1.Opening1.Button_detection.Timer_LL [order 1] : [not(FLAG_STOP)]
          OpCl_doors.OpCl_1.Opening1.Button_detection.Timer_LL -> OpCl_doors.OpCl_1.Opening1.Button_detection.Save_energy
          OpCl_doors.OpCl_1.Opening1.Button_detection.Save_energy -> (junction 88388)
          (junction 88386) -> (junction 88389) [order 2]
          (junction 88387) -> (junction 88390) [order 2]
          (junction 88388) -> (junction 88391)
          (junction 88390) -> (junction 88389)
          (junction 88391) -> (junction 88390)
          (junction 88389) -> OpCl_doors.OpCl_1.Opening1.Button_detection.BUTTON_CAR
          OpCl_doors.OpCl_1.Opening1.Button_detection.BUTTON_UP -> OpCl_doors.OpCl_1.Opening1.Button_detection.BUTTON_DOWN
          OpCl_doors.OpCl_1.Opening1.Button_detection.BUTTON_DOWN -> OpCl_doors.OpCl_1.Opening1.Button_detection.Max_Min_assignment
          OpCl_doors.OpCl_1.Opening1.Button_detection.Max_Min_assignment -> (junction 88392)
          OpCl_doors.OpCl_1.Opening1.Button_detection.BUTTON_CAR -> OpCl_doors.OpCl_1.Opening1.Button_detection.BUTTON_UP
          (junction 88392) -> (junction 88394)
          (junction 88394) -> (junction 88393)
          (junction 88393) -> (junction 88395)
          (junction 88395) -> (junction 88396) [order 1] : [FLAG==1]
          (junction 88396) -> OpCl_doors.OpCl_1.Opening1.Button_detection.GoTo_PositionControl [order 1] : [PUSHED]
          OpCl_doors.OpCl_1.Opening1.Button_detection.GoTo_PositionControl -> (junction 88397)
          (junction 88395) -> (junction 88407) [order 2]
          (junction 88396) -> (junction 88398) [order 2]
          (junction 88397) -> (junction 88399)
          (junction 88399) -> (junction 88398)
          (junction 88398) -> (junction 88401)
          OpCl_doors.OpCl_1.Opening1.Button_detection.Emergency -> (junction 88400)
          (junction 88401) -> OpCl_doors.OpCl_1.Opening1.Button_detection.Timer_EME [order 1] : [STOP]
              | {IN_LL=false; ET_LL=0;FLAG=1;}
          OpCl_doors.OpCl_1.Opening1.Button_detection.Timer_EME -> (junction 88402)
          (junction 88402) -> OpCl_doors.OpCl_1.Opening1.Button_detection.Emergency [order 1] : [Q_EME]
          (junction 88400) -> (junction 88404)
          (junction 88401) -> OpCl_doors.OpCl_1.Opening1.Button_detection.Not_Emergency [order 2]
          (junction 88402) -> (junction 88403) [order 2]
          (junction 88404) -> (junction 88403)
          (junction 88403) -> (junction 88406)
          OpCl_doors.OpCl_1.Opening1.Button_detection.Not_Emergency -> (junction 88406)
          OpCl_doors.OpCl_1.Opening1.Button_detection.SwitchingOFF_LEDs -> (junction 88405)
          (junction 88406) -> OpCl_doors.OpCl_1.Opening1.Button_detection.SwitchingOFF_LEDs [order 1] : [FLAG_STOP && FLAG==2]
          (junction 88405) -> (junction 88409)
          (junction 88406) -> (junction 88408) [order 2]
          (junction 88408) -> (junction 88407)
          (junction 88409) -> (junction 88408)
        state Button_detection1
          state Save_energy
            en:
            LL=not(Q_LL);
          state Timer_LL
            state Set_tmr
              en:
              Q_LL=true;
            state Counting
              en:
              ET_LL= ET_LL + 1;
              Q_LL=false;
            state Set
              en:
              IN_LL=true;
              PT_LL=10;
            (junction 88870) -> OpCl_doors.OpCl_1.Opening1.Button_detection1.Timer_LL.Set_tmr [order 1] : [ET_LL==PT_LL]
            OpCl_doors.OpCl_1.Opening1.Button_detection1.Timer_LL.Set_tmr -> (junction 88871)
            OpCl_doors.OpCl_1.Opening1.Button_detection1.Timer_LL.Counting -> (junction 88870)
            (junction 88870) -> (junction 88871) [order 2]
            (default) -> OpCl_doors.OpCl_1.Opening1.Button_detection1.Timer_LL.Set
            OpCl_doors.OpCl_1.Opening1.Button_detection1.Timer_LL.Set -> (junction 88872)
            (junction 88872) -> OpCl_doors.OpCl_1.Opening1.Button_detection1.Timer_LL.Counting [order 1] : [ET_LL<PT_LL]
            (junction 88872) -> (junction 88871) [order 2]
          state BUTTON_DOWN
            state Button_DOWN_1
              en:
              BUTTON_DOWN(2)=true;
              BUT_TEMP=1;
              LPD1=true;
              PUSHED=true;
              UPDATE=false;
              IN_LL=false; ET_LL=0;
            state First_but_1
              en:
              BUT_1=BUT_TEMP;
              FIRST_BUT=false;
            state Button_DOWN_2
              en:
              BUTTON_DOWN(3)=true;
              BUT_TEMP=2;
              LPD2=true;
              PUSHED=true;
              UPDATE=false;
              IN_LL=false; ET_LL=0;
            state First_but_2
              en:
              BUT_1=BUT_TEMP;
              FIRST_BUT=false;
            state Button_DOWN_3
              en:
              BUTTON_DOWN(4)=true;
              BUT_TEMP=3;
              LPD3=true;
              PUSHED=true;
              UPDATE=false;
              IN_LL=false; ET_LL=0;
            state First_but_3
              en:
              BUT_1=BUT_TEMP;
              FIRST_BUT=false;
            (default) -> (junction 88885)
            (junction 88885) -> OpCl_doors.OpCl_1.Opening1.Button_detection1.BUTTON_DOWN.Button_DOWN_1 [order 1] : [PD1]
            OpCl_doors.OpCl_1.Opening1.Button_detection1.BUTTON_DOWN.Button_DOWN_1 -> (junction 88886)
            (junction 88886) -> OpCl_doors.OpCl_1.Opening1.Button_detection1.BUTTON_DOWN.First_but_1 [order 1] : [FIRST_BUT && not(RPC1)]
            OpCl_doors.OpCl_1.Opening1.Button_detection1.BUTTON_DOWN.First_but_1 -> (junction 88887)
            (junction 88885) -> (junction 88888) [order 2]
            (junction 88886) -> (junction 88889) [order 2]
            (junction 88887) -> (junction 88890)
            (junction 88889) -> (junction 88888)
            (junction 88890) -> (junction 88889)
            (junction 88888) -> (junction 88891)
            (junction 88891) -> OpCl_doors.OpCl_1.Opening1.Button_detection1.BUTTON_DOWN.Button_DOWN_2 [order 1] : [PD2]
            OpCl_doors.OpCl_1.Opening1.Button_detection1.BUTTON_DOWN.Button_DOWN_2 -> (junction 88892)
            (junction 88892) -> OpCl_doors.OpCl_1.Opening1.Button_detection1.BUTTON_DOWN.First_but_2 [order 1] : [FIRST_BUT && not(RPC2)]
            OpCl_doors.OpCl_1.Opening1.Button_detection1.BUTTON_DOWN.First_but_2 -> (junction 88893)
            (junction 88891) -> (junction 88894) [order 2]
            (junction 88892) -> (junction 88895) [order 2]
            (junction 88893) -> (junction 88896)
            (junction 88895) -> (junction 88894)
            (junction 88896) -> (junction 88895)
            (junction 88894) -> (junction 88897)
            (junction 88897) -> OpCl_doors.OpCl_1.Opening1.Button_detection1.BUTTON_DOWN.Button_DOWN_3 [order 1] : [PD3]
            OpCl_doors.OpCl_1.Opening1.Button_detection1.BUTTON_DOWN.Button_DOWN_3 -> (junction 88898)
            (junction 88898) -> OpCl_doors.OpCl_1.Opening1.Button_detection1.BUTTON_DOWN.First_but_3 [order 1] : [FIRST_BUT && not(RPC3)]
            OpCl_doors.OpCl_1.Opening1.Button_detection1.BUTTON_DOWN.First_but_3 -> (junction 88899)
            (junction 88897) -> (junction 88900) [order 2]
            (junction 88898) -> (junction 88901) [order 2]
            (junction 88899) -> (junction 88902)
            (junction 88901) -> (junction 88900)
            (junction 88902) -> (junction 88901)
          state BUTTON_CAR
            state Button_CAR_0
              en:
              BUTTON_CAR(1)=true;
              BUT_TEMP=0;
              LPC0=true;
              PUSHED=true;
              UPDATE=false;
              IN_LL=false; ET_LL=0;
            state First_but_0
              en:
              BUT_1=BUT_TEMP;
              FIRST_BUT=false;
            state Button_CAR_1
              en:
              BUTTON_CAR(2)=true;
              BUT_TEMP=1;
              LPC1=true;
              PUSHED=true;
              UPDATE=false;
              IN_LL=false; ET_LL=0;
            state First_but_1
              en:
              BUT_1=BUT_TEMP;
              FIRST_BUT=false;
            state Button_CAR_2
              en:
              BUTTON_CAR(3)=true;
              BUT_TEMP=2;
              LPC2=true;
              PUSHED=true;
              UPDATE=false;
              IN_LL=false; ET_LL=0;
            state First_but_2
              en:
              BUT_1=BUT_TEMP;
              FIRST_BUT=false;
            state Button_CAR_3
              en:
              BUTTON_CAR(4)=true;
              BUT_TEMP=3;
              LPC3=true;
              PUSHED=true;
              UPDATE=false;
              IN_LL=false; ET_LL=0;
            state First_but_3
              en:
              BUT_1=BUT_TEMP;
              FIRST_BUT=false;
            (default) -> (junction 88940)
            (junction 88940) -> OpCl_doors.OpCl_1.Opening1.Button_detection1.BUTTON_CAR.Button_CAR_0 [order 1] : [P0]
            OpCl_doors.OpCl_1.Opening1.Button_detection1.BUTTON_CAR.Button_CAR_0 -> (junction 88941)
            (junction 88941) -> OpCl_doors.OpCl_1.Opening1.Button_detection1.BUTTON_CAR.First_but_0 [order 1] : [FIRST_BUT && not(RPC0)]
            OpCl_doors.OpCl_1.Opening1.Button_detection1.BUTTON_CAR.First_but_0 -> (junction 88942)
            (junction 88940) -> (junction 88943) [order 2]
            (junction 88941) -> (junction 88944) [order 2]
            (junction 88942) -> (junction 88945)
            (junction 88944) -> (junction 88943)
            (junction 88945) -> (junction 88944)
            (junction 88943) -> (junction 88948)
            OpCl_doors.OpCl_1.Opening1.Button_detection1.BUTTON_CAR.Button_CAR_1 -> (junction 88946)
            (junction 88946) -> OpCl_doors.OpCl_1.Opening1.Button_detection1.BUTTON_CAR.First_but_1 [order 1] : [FIRST_BUT && not(RPC1)]
            OpCl_doors.OpCl_1.Opening1.Button_detection1.BUTTON_CAR.First_but_1 -> (junction 88947)
            (junction 88946) -> (junction 88950) [order 2]
            (junction 88947) -> (junction 88951)
            (junction 88948) -> OpCl_doors.OpCl_1.Opening1.Button_detection1.BUTTON_CAR.Button_CAR_1 [order 1] : [P1]
            (junction 88948) -> (junction 88949) [order 2]
            (junction 88950) -> (junction 88949)
            (junction 88951) -> (junction 88950)
            (junction 88949) -> (junction 88952)
            (junction 88952) -> OpCl_doors.OpCl_1.Opening1.Button_detection1.BUTTON_CAR.Button_CAR_2 [order 1] : [P2]
            OpCl_doors.OpCl_1.Opening1.Button_detection1.BUTTON_CAR.Button_CAR_2 -> (junction 88953)
            (junction 88953) -> OpCl_doors.OpCl_1.Opening1.Button_detection1.BUTTON_CAR.First_but_2 [order 1] : [FIRST_BUT && not(RPC2)]
            OpCl_doors.OpCl_1.Opening1.Button_detection1.BUTTON_CAR.First_but_2 -> (junction 88954)
            (junction 88952) -> (junction 88955) [order 2]
            (junction 88953) -> (junction 88956) [order 2]
            (junction 88954) -> (junction 88957)
            (junction 88956) -> (junction 88955)
            (junction 88957) -> (junction 88956)
            (junction 88955) -> (junction 88958)
            (junction 88958) -> OpCl_doors.OpCl_1.Opening1.Button_detection1.BUTTON_CAR.Button_CAR_3 [order 1] : [P3]
            OpCl_doors.OpCl_1.Opening1.Button_detection1.BUTTON_CAR.Button_CAR_3 -> (junction 88959)
            (junction 88959) -> OpCl_doors.OpCl_1.Opening1.Button_detection1.BUTTON_CAR.First_but_3 [order 1] : [FIRST_BUT && not(RPC3)]
            OpCl_doors.OpCl_1.Opening1.Button_detection1.BUTTON_CAR.First_but_3 -> (junction 88960)
            (junction 88958) -> (junction 88961) [order 2]
            (junction 88959) -> (junction 88962) [order 2]
            (junction 88960) -> (junction 88963)
            (junction 88962) -> (junction 88961)
            (junction 88963) -> (junction 88962)
          state BUTTON_UP
            state Button_UP_0
              en:
              BUTTON_UP(1)=true;
              BUT_TEMP=0;
              LPS0=true;
              PUSHED=true;
              UPDATE=false;
              IN_LL=false; ET_LL=0;
            state First_but_0
              en:
              BUT_1=BUT_TEMP;
              FIRST_BUT=false;
            state Button_UP_1
              en:
              BUTTON_UP(2)=true;
              BUT_TEMP=1;
              LPS1=true;
              PUSHED=true;
              UPDATE=false;
              IN_LL=false; ET_LL=0;
            state First_but_1
              en:
              BUT_1=BUT_TEMP;
              FIRST_BUT=false;
            state Button_UP_2
              en:
              BUTTON_UP(3)=true;
              BUT_TEMP=2;
              LPS2=true;
              PUSHED=true;
              UPDATE=false;
              IN_LL=false; ET_LL=0;
            state First_but_2
              en:
              BUT_1=BUT_TEMP;
              FIRST_BUT=false;
            (junction 89013) -> OpCl_doors.OpCl_1.Opening1.Button_detection1.BUTTON_UP.Button_UP_0 [order 1] : [PS0]
            OpCl_doors.OpCl_1.Opening1.Button_detection1.BUTTON_UP.Button_UP_0 -> (junction 89014)
            (junction 89014) -> OpCl_doors.OpCl_1.Opening1.Button_detection1.BUTTON_UP.First_but_0 [order 1] : [FIRST_BUT && not(RPC0)]
            OpCl_doors.OpCl_1.Opening1.Button_detection1.BUTTON_UP.First_but_0 -> (junction 89015)
            (default) -> (junction 89013)
            (junction 89013) -> (junction 89018) [order 2]
            (junction 89014) -> (junction 89016) [order 2]
            (junction 89015) -> (junction 89017)
            (junction 89017) -> (junction 89016)
            (junction 89016) -> (junction 89018)
            (junction 89018) -> (junction 89019)
            (junction 89019) -> OpCl_doors.OpCl_1.Opening1.Button_detection1.BUTTON_UP.Button_UP_1 [order 1] : [PS1]
            OpCl_doors.OpCl_1.Opening1.Button_detection1.BUTTON_UP.Button_UP_1 -> (junction 89020)
            (junction 89020) -> OpCl_doors.OpCl_1.Opening1.Button_detection1.BUTTON_UP.First_but_1 [order 1] : [FIRST_BUT && not(RPC1)]
            OpCl_doors.OpCl_1.Opening1.Button_detection1.BUTTON_UP.First_but_1 -> (junction 89021)
            (junction 89019) -> (junction 89022) [order 2]
            (junction 89020) -> (junction 89023) [order 2]
            (junction 89021) -> (junction 89024)
            (junction 89023) -> (junction 89022)
            (junction 89024) -> (junction 89023)
            (junction 89022) -> (junction 89026)
            OpCl_doors.OpCl_1.Opening1.Button_detection1.BUTTON_UP.First_but_2 -> (junction 89025)
            (junction 89025) -> (junction 89030)
            (junction 89026) -> OpCl_doors.OpCl_1.Opening1.Button_detection1.BUTTON_UP.Button_UP_2 [order 1] : [PS2]
            OpCl_doors.OpCl_1.Opening1.Button_detection1.BUTTON_UP.Button_UP_2 -> (junction 89027)
            (junction 89027) -> OpCl_doors.OpCl_1.Opening1.Button_detection1.BUTTON_UP.First_but_2 [order 1] : [FIRST_BUT && not(RPC2)]
            (junction 89026) -> (junction 89028) [order 2]
            (junction 89027) -> (junction 89029) [order 2]
            (junction 89029) -> (junction 89028)
            (junction 89030) -> (junction 89029)
          state Max_Min_assignment
            state Min_but
              en:
              BUTTON=MIN_BUT;
            state Max_but
              en:
              BUTTON=MAX_BUT;
            state First_but
              en:
              BUTTON=BUT_1;
            state Max_but1
              en:
              MAX_BUT=2;
            state Max_but2
              en:
              MAX_BUT=1;
            state Max_but3
              en:
              MAX_BUT=0;
            state Min_but1
              en:
              MIN_BUT=1;
            state Min_but2
              en:
              MIN_BUT=2;
            state Min_but3
              en:
              MIN_BUT=3;
            state MAX
              en:
              MAX_BUT=BUT_TEMP;
            state MIN
              en:
              MIN_BUT=BUT_TEMP;
            state Updating_button_0
              en:
              BUTTON=MAX_BUT;
            state Updating_button_1
              en:
              BUTTON=MIN_BUT;
            (junction 89068) -> OpCl_doors.OpCl_1.Opening1.Button_detection1.Max_Min_assignment.Min_but [order 1] : [(MAX_BUT-FLOOR)>(FLOOR-MIN_BUT)]
            OpCl_doors.OpCl_1.Opening1.Button_detection1.Max_Min_assignment.Min_but -> (junction 89069)
            (junction 89070) -> (junction 89068) [order 1] : [not(FLAG_STOP) && MOTION==2 && FLAG==3]
            (default) -> (junction 89070)
            (junction 89068) -> (junction 89071) [order 2]
            (junction 89069) -> (junction 89072)
            (junction 89070) -> (junction 89073) [order 2]
            (junction 89071) -> OpCl_doors.OpCl_1.Opening1.Button_detection1.Max_Min_assignment.Max_but [order 1] : [(MAX_BUT-FLOOR)<(FLOOR-MIN_BUT)]
            OpCl_doors.OpCl_1.Opening1.Button_detection1.Max_Min_assignment.Max_but -> (junction 89072)
            (junction 89071) -> OpCl_doors.OpCl_1.Opening1.Button_detection1.Max_Min_assignment.First_but [order 2]
            (junction 89072) -> (junction 89075)
            OpCl_doors.OpCl_1.Opening1.Button_detection1.Max_Min_assignment.First_but -> (junction 89074)
            (junction 89074) -> (junction 89073)
            (junction 89075) -> (junction 89074)
            (junction 89073) -> (junction 89076)
            (junction 89077) -> (junction 89078) [order 1] : [MOTION==0]
                | {MOTION=1;
                | UPDATE=true;}
            (junction 89078) -> OpCl_doors.OpCl_1.Opening1.Button_detection1.Max_Min_assignment.Max_but1 [order 1] : [BUTTON_UP(2)]
            OpCl_doors.OpCl_1.Opening1.Button_detection1.Max_Min_assignment.Max_but1 -> (junction 89079)
            (junction 89076) -> (junction 89077) [order 1] : [BUTTON==FLOOR && EXTEND]
                | {EXTEND=false;}
            (junction 89076) -> (junction 89090) [order 2]
            (junction 89077) -> (junction 89082) [order 2]
            (junction 89078) -> (junction 89080) [order 2]
            (junction 89079) -> (junction 89081)
            (junction 89080) -> OpCl_doors.OpCl_1.Opening1.Button_detection1.Max_Min_assignment.Max_but2 [order 1] : [BUTTON_UP(1)]
            OpCl_doors.OpCl_1.Opening1.Button_detection1.Max_Min_assignment.Max_but2 -> (junction 89081)
            (junction 89080) -> OpCl_doors.OpCl_1.Opening1.Button_detection1.Max_Min_assignment.Max_but3 [order 2]
            (junction 89081) -> (junction 89084)
            OpCl_doors.OpCl_1.Opening1.Button_detection1.Max_Min_assignment.Max_but3 -> (junction 89083)
            (junction 89083) -> (junction 89082)
            (junction 89084) -> (junction 89083)
            (junction 89082) -> (junction 89085)
            (junction 89085) -> (junction 89086) [order 1] : [MOTION==1]
                | {MOTION=0;
                | UPDATE=true;}
            (junction 89086) -> OpCl_doors.OpCl_1.Opening1.Button_detection1.Max_Min_assignment.Min_but1 [order 1] : [BUTTON_DOWN(1)]
            OpCl_doors.OpCl_1.Opening1.Button_detection1.Max_Min_assignment.Min_but1 -> (junction 89087)
            (junction 89085) -> (junction 89091) [order 2]
            (junction 89086) -> (junction 89088) [order 2]
            (junction 89087) -> (junction 89089)
            (junction 89088) -> OpCl_doors.OpCl_1.Opening1.Button_detection1.Max_Min_assignment.Min_but2 [order 1] : [BUTTON_DOWN(2)]
            OpCl_doors.OpCl_1.Opening1.Button_detection1.Max_Min_assignment.Min_but2 -> (junction 89089)
            (junction 89088) -> OpCl_doors.OpCl_1.Opening1.Button_detection1.Max_Min_assignment.Min_but3 [order 2]
            (junction 89089) -> (junction 89093)
            OpCl_doors.OpCl_1.Opening1.Button_detection1.Max_Min_assignment.Min_but3 -> (junction 89092)
            (junction 89091) -> (junction 89090)
            (junction 89092) -> (junction 89091)
            (junction 89093) -> (junction 89092)
            (junction 89090) -> (junction 89095)
            OpCl_doors.OpCl_1.Opening1.Button_detection1.Max_Min_assignment.MAX -> (junction 89094)
            (junction 89095) -> (junction 89096) [order 1] : [PUSHED]
            (junction 89096) -> (junction 89097) [order 1] : [not(BUT_TEMP==FLOOR) || not(MOTION==2)]
            (junction 89097) -> OpCl_doors.OpCl_1.Opening1.Button_detection1.Max_Min_assignment.MAX [order 1] : [MAX_BUT<BUT_TEMP && not(UPDATE)]
            (junction 89094) -> (junction 89099)
            (junction 89095) -> (junction 89109) [order 2]
            (junction 89096) -> (junction 89102) [order 2]
            (junction 89097) -> (junction 89098) [order 2]
            (junction 89099) -> (junction 89098)
            (junction 89098) -> (junction 89100)
            (junction 89100) -> OpCl_doors.OpCl_1.Opening1.Button_detection1.Max_Min_assignment.MIN [order 1] : [MIN_BUT>BUT_TEMP && not(UPDATE)]
            OpCl_doors.OpCl_1.Opening1.Button_detection1.Max_Min_assignment.MIN -> (junction 89101)
            (junction 89100) -> (junction 89103) [order 2]
            (junction 89101) -> (junction 89104)
            (junction 89103) -> (junction 89102)
            (junction 89104) -> (junction 89103)
            (junction 89102) -> (junction 89105)
            (junction 89105) -> OpCl_doors.OpCl_1.Opening1.Button_detection1.Max_Min_assignment.Updating_button_0 [order 1] : [MOTION==0]
            OpCl_doors.OpCl_1.Opening1.Button_detection1.Max_Min_assignment.Updating_button_0 -> (junction 89106)
            (junction 89105) -> (junction 89107) [order 2]
            (junction 89106) -> (junction 89108)
            (junction 89107) -> OpCl_doors.OpCl_1.Opening1.Button_detection1.Max_Min_assignment.Updating_button_1 [order 1] : [MOTION==1]
            OpCl_doors.OpCl_1.Opening1.Button_detection1.Max_Min_assignment.Updating_button_1 -> (junction 89108)
            (junction 89107) -> (junction 89110) [order 2]
            (junction 89108) -> (junction 89111)
            (junction 89110) -> (junction 89109)
            (junction 89111) -> (junction 89110)
          state GoTo_PositionControl
            en:
            BUTTON=BUT_TEMP;
            FLAG=2;
          state Emergency
            en:
            FLAG_EMG=true;
            FLAG=4;
          state Timer_EME
            state Set_tmr
              en:
              Q_EME=true;
            state Counting
              en:
              ET_EME= ET_EME + 1;
              Q_EME=false;
            state Set
              en:
              IN_EME=true;
              PT_EME=3;
            (junction 89201) -> OpCl_doors.OpCl_1.Opening1.Button_detection1.Timer_EME.Set_tmr [order 1] : [ET_EME==PT_EME]
            OpCl_doors.OpCl_1.Opening1.Button_detection1.Timer_EME.Set_tmr -> (junction 89202)
            OpCl_doors.OpCl_1.Opening1.Button_detection1.Timer_EME.Counting -> (junction 89201)
            (junction 89201) -> (junction 89202) [order 2]
            (default) -> OpCl_doors.OpCl_1.Opening1.Button_detection1.Timer_EME.Set
            OpCl_doors.OpCl_1.Opening1.Button_detection1.Timer_EME.Set -> (junction 89203)
            (junction 89203) -> OpCl_doors.OpCl_1.Opening1.Button_detection1.Timer_EME.Counting [order 1] : [ET_EME<PT_EME]
            (junction 89203) -> (junction 89202) [order 2]
          state Not_Emergency
            en:
            IN_EME=false;
            ET_EME=0;
          state SwitchingOFF_LEDs
            en:
            LPD3=false;
            LPD2=false;
            LPS2=false;
            LPD1=false;
            LPS1=false;
            LPS0=false;
          (default) -> (junction 88802)
          (junction 88802) -> (junction 88803) [order 1] : [FLAG==1 && not(PUSHED)]
              | {BUTTON=FLOOR;
              | BUT_TEMP=BUTTON;
              | BUT_1=FLOOR;}
          (junction 88803) -> OpCl_doors.OpCl_1.Opening1.Button_detection1.Timer_LL [order 1] : [not(FLAG_STOP)]
          OpCl_doors.OpCl_1.Opening1.Button_detection1.Save_energy -> (junction 88804)
          OpCl_doors.OpCl_1.Opening1.Button_detection1.Timer_LL -> OpCl_doors.OpCl_1.Opening1.Button_detection1.Save_energy
          (junction 88803) -> (junction 88806) [order 2]
          (junction 88802) -> (junction 88805) [order 2]
          (junction 88804) -> (junction 88807)
          (junction 88806) -> (junction 88805)
          (junction 88807) -> (junction 88806)
          (junction 88805) -> OpCl_doors.OpCl_1.Opening1.Button_detection1.BUTTON_CAR
          OpCl_doors.OpCl_1.Opening1.Button_detection1.BUTTON_UP -> OpCl_doors.OpCl_1.Opening1.Button_detection1.BUTTON_DOWN
          OpCl_doors.OpCl_1.Opening1.Button_detection1.BUTTON_DOWN -> OpCl_doors.OpCl_1.Opening1.Button_detection1.Max_Min_assignment
          OpCl_doors.OpCl_1.Opening1.Button_detection1.Max_Min_assignment -> (junction 88808)
          OpCl_doors.OpCl_1.Opening1.Button_detection1.BUTTON_CAR -> OpCl_doors.OpCl_1.Opening1.Button_detection1.BUTTON_UP
          (junction 88808) -> (junction 88810)
          (junction 88810) -> (junction 88809)
          (junction 88809) -> (junction 88812)
          OpCl_doors.OpCl_1.Opening1.Button_detection1.GoTo_PositionControl -> (junction 88811)
          (junction 88812) -> (junction 88813) [order 1] : [FLAG==1]
          (junction 88813) -> OpCl_doors.OpCl_1.Opening1.Button_detection1.GoTo_PositionControl [order 1] : [PUSHED]
          (junction 88811) -> (junction 88815)
          (junction 88812) -> (junction 88823) [order 2]
          (junction 88813) -> (junction 88814) [order 2]
          (junction 88815) -> (junction 88814)
          (junction 88814) -> (junction 88817)
          OpCl_doors.OpCl_1.Opening1.Button_detection1.Emergency -> (junction 88816)
          (junction 88817) -> OpCl_doors.OpCl_1.Opening1.Button_detection1.Timer_EME [order 1] : [STOP]
              | {IN_LL=false; ET_LL=0;FLAG=1;}
          OpCl_doors.OpCl_1.Opening1.Button_detection1.Timer_EME -> (junction 88818)
          (junction 88818) -> OpCl_doors.OpCl_1.Opening1.Button_detection1.Emergency [order 1] : [Q_EME]
          (junction 88816) -> (junction 88820)
          (junction 88817) -> OpCl_doors.OpCl_1.Opening1.Button_detection1.Not_Emergency [order 2]
          (junction 88818) -> (junction 88819) [order 2]
          (junction 88820) -> (junction 88819)
          (junction 88819) -> (junction 88822)
          OpCl_doors.OpCl_1.Opening1.Button_detection1.Not_Emergency -> (junction 88822)
          OpCl_doors.OpCl_1.Opening1.Button_detection1.SwitchingOFF_LEDs -> (junction 88821)
          (junction 88822) -> OpCl_doors.OpCl_1.Opening1.Button_detection1.SwitchingOFF_LEDs [order 1] : [FLAG_STOP && FLAG==2]
          (junction 88821) -> (junction 88825)
          (junction 88822) -> (junction 88824) [order 2]
          (junction 88824) -> (junction 88823)
          (junction 88825) -> (junction 88824)
        state Opening1
          en:AP1=true;
        state Reset
          state Reset_0
            en:
            LPS0=false;
            BUTTON_CAR(1)=false;
            BUTTON_UP(1)=false;
          state Reset_1
            en:
            LPS1=false;
            LPD1=false;
            BUTTON_CAR(2)=false;
            BUTTON_UP(2)=false;
            BUTTON_DOWN(2)=false;
          state Reset_2
            en:
            LPS2=false;
            LPD2=false;
            BUTTON_CAR(3)=false;
            BUTTON_UP(3)=false;
            BUTTON_DOWN(3)=false;
          state Reset_3
            en:
            LPD3=false;
            BUTTON_CAR(4)=false;
            BUTTON_DOWN(4)=false;
          (default) -> (junction 89219)
          (junction 89219) -> OpCl_doors.OpCl_1.Opening1.Reset.Reset_0 [order 1] : [FLOOR==0]
          OpCl_doors.OpCl_1.Opening1.Reset.Reset_0 -> (junction 89220)
          (junction 89219) -> (junction 89221) [order 2]
          (junction 89220) -> (junction 89222)
          (junction 89221) -> OpCl_doors.OpCl_1.Opening1.Reset.Reset_1 [order 1] : [FLOOR==1]
          OpCl_doors.OpCl_1.Opening1.Reset.Reset_1 -> (junction 89222)
          (junction 89221) -> (junction 89223) [order 2]
          (junction 89222) -> (junction 89224)
          (junction 89223) -> OpCl_doors.OpCl_1.Opening1.Reset.Reset_2 [order 1] : [FLOOR==2]
          OpCl_doors.OpCl_1.Opening1.Reset.Reset_2 -> (junction 89224)
          (junction 89223) -> (junction 89225) [order 2]
          (junction 89224) -> (junction 89226)
          (junction 89225) -> OpCl_doors.OpCl_1.Opening1.Reset.Reset_3 [order 1] : [FLOOR==3]
          OpCl_doors.OpCl_1.Opening1.Reset.Reset_3 -> (junction 89226)
          (junction 89225) -> (junction 89227) [order 2]
          (junction 89226) -> (junction 89228)
          (junction 89228) -> (junction 89227)
        state Stop_Opening1
          en: AP1=false;
          FLAG_OD=true;
          IN_cl=false;
          ET_cl=0;
        (junction 88216) -> (junction 88217)
        (junction 88217) -> (junction 88218) [order 1] : [not(OBS) ]
        (junction 88220) -> OpCl_doors.OpCl_1.Opening1.Opening [order 1] : [not(PA1)]
        (junction 88218) -> (junction 88219) [order 2]
        (junction 88219) -> OpCl_doors.OpCl_1.Opening1.Timer_open
        OpCl_doors.OpCl_1.Opening1.Timer_open -> (junction 88220)
        (default) -> OpCl_doors.OpCl_1.Opening1.People_IN
        (junction 88217) -> (junction 88221) [order 2]
        (junction 88218) -> OpCl_doors.OpCl_1.Opening1.Button_detection [order 1] : [not(FLAG==4)]
        (junction 88223) -> (junction 88219)
        (junction 88225) -> (junction 88216)
        (junction 88220) -> OpCl_doors.OpCl_1.Opening1.Stop_Opening [order 2]
        OpCl_doors.OpCl_1.Opening1.People_IN -> OpCl_doors.OpCl_1.Opening1.People_OUT
        OpCl_doors.OpCl_1.Opening1.Opening -> (junction 88230)
        (junction 88221) -> (junction 88222) [order 2]
        (junction 88221) -> OpCl_doors.OpCl_1.Opening1.Button_detection1 [order 1] : [not(FLAG==4)]
        (junction 88222) -> (junction 88227)
        OpCl_doors.OpCl_1.Opening1.Button_detection -> (junction 88223)
        OpCl_doors.OpCl_1.Opening1.People_OUT -> (junction 88224)
        OpCl_doors.OpCl_1.Opening1.Button_detection1 -> (junction 88226)
        (junction 88227) -> (junction 88226)
        (junction 88224) -> (junction 88225) [order 2]
        (junction 88224) -> OpCl_doors.OpCl_1.Opening1.Reset [order 1] : [not(FLAG==4)]
        (junction 88226) -> (junction 88228)
        (junction 88234) -> (junction 88225)
        OpCl_doors.OpCl_1.Opening1.Stop_Opening -> (junction 88229)
        (junction 88228) -> OpCl_doors.OpCl_1.Opening1.Opening1 [order 1] : [not(PA1)]
        (junction 88228) -> OpCl_doors.OpCl_1.Opening1.Stop_Opening1 [order 2]
        (junction 88230) -> (junction 88229)
        (junction 88229) -> (junction 88232)
        OpCl_doors.OpCl_1.Opening1.Opening1 -> (junction 88231)
        OpCl_doors.OpCl_1.Opening1.Reset -> (junction 88233)
        OpCl_doors.OpCl_1.Opening1.Stop_Opening1 -> (junction 88231)
        (junction 88231) -> (junction 88232)
        (junction 88233) -> (junction 88234)
      (default) -> (junction 12692)
      (junction 12692) -> (junction 12691) [order 1] : [FLAG_OD]
      (junction 12691) -> OpCl_doors.OpCl_1.Closing1 [order 1] : [not(SWITCH) && not(STOP) && WEIGHT<=320 && not(PS1 || PD1 || P1)]
      OpCl_doors.OpCl_1.Closing1 -> (junction 30477)
      (junction 12692) -> OpCl_doors.OpCl_1.Opening1 [order 2]
      (junction 12691) -> OpCl_doors.OpCl_1.StopClosing [order 2]
      (junction 30477) -> (junction 30480)
      OpCl_doors.OpCl_1.StopClosing -> (junction 30478)
      (junction 30480) -> (junction 30478)
      (junction 30478) -> (junction 30484)
      OpCl_doors.OpCl_1.Opening1 -> (junction 30484)
    state OpCl_2
      state Closing2
        state Reset
          state Reset_0
            en:
            LPS0=false;
            BUTTON_CAR(1)=false;
            BUTTON_UP(1)=false;
          state Reset_1
            en:
            LPS1=false;
            LPD1=false;
            BUTTON_CAR(2)=false;
            BUTTON_UP(2)=false;
            BUTTON_DOWN(2)=false;
          state Reset_2
            en:
            LPS2=false;
            LPD2=false;
            BUTTON_CAR(3)=false;
            BUTTON_UP(3)=false;
            BUTTON_DOWN(3)=false;
          state Reset_3
            en:
            LPD3=false;
            BUTTON_CAR(4)=false;
            BUTTON_DOWN(4)=false;
          (default) -> (junction 69957)
          (junction 69957) -> OpCl_doors.OpCl_2.Closing2.Reset.Reset_0 [order 1] : [FLOOR==0]
          OpCl_doors.OpCl_2.Closing2.Reset.Reset_0 -> (junction 69958)
          (junction 69957) -> (junction 69959) [order 2]
          (junction 69958) -> (junction 69960)
          (junction 69959) -> OpCl_doors.OpCl_2.Closing2.Reset.Reset_1 [order 1] : [FLOOR==1]
          OpCl_doors.OpCl_2.Closing2.Reset.Reset_1 -> (junction 69960)
          (junction 69959) -> (junction 69961) [order 2]
          (junction 69960) -> (junction 69962)
          (junction 69961) -> OpCl_doors.OpCl_2.Closing2.Reset.Reset_2 [order 1] : [FLOOR==2]
          OpCl_doors.OpCl_2.Closing2.Reset.Reset_2 -> (junction 69962)
          (junction 69961) -> (junction 69963) [order 2]
          (junction 69962) -> (junction 69964)
          (junction 69963) -> OpCl_doors.OpCl_2.Closing2.Reset.Reset_3 [order 1] : [FLOOR==3]
          OpCl_doors.OpCl_2.Closing2.Reset.Reset_3 -> (junction 69964)
          (junction 69963) -> (junction 69965) [order 2]
          (junction 69964) -> (junction 69966)
          (junction 69966) -> (junction 69965)
        state Timer_close
          state Set_tmr
            en: Q_cl=true;
          state Set
            en:PT_cl=5;
            IN_cl=true;
          state Counting
            en:ET_cl = ET_cl + 1;
            Q_cl=false;
          (junction 69990) -> OpCl_doors.OpCl_2.Closing2.Timer_close.Set_tmr [order 1] : [ET_cl==PT_cl]
          OpCl_doors.OpCl_2.Closing2.Timer_close.Set_tmr -> (junction 69991)
          (default) -> OpCl_doors.OpCl_2.Closing2.Timer_close.Set
          OpCl_doors.OpCl_2.Closing2.Timer_close.Counting -> (junction 69990)
          (junction 69990) -> (junction 69991) [order 2]
          OpCl_doors.OpCl_2.Closing2.Timer_close.Set -> (junction 69992)
          (junction 69992) -> OpCl_doors.OpCl_2.Closing2.Timer_close.Counting [order 1] : [ET_cl<PT_cl]
          (junction 69992) -> (junction 69991) [order 2]
        state Closing
          en: CP2=Q_cl;
        state Button_detection
          state Save_energy
            en:
            LL=not(Q_LL);
          state Timer_LL
            state Set_tmr
              en:
              Q_LL=true;
            state Counting
              en:
              ET_LL= ET_LL + 1;
              Q_LL=false;
            state Set
              en:
              IN_LL=true;
              PT_LL=10;
            (junction 70074) -> OpCl_doors.OpCl_2.Closing2.Button_detection.Timer_LL.Set_tmr [order 1] : [ET_LL==PT_LL]
            OpCl_doors.OpCl_2.Closing2.Button_detection.Timer_LL.Set_tmr -> (junction 70075)
            OpCl_doors.OpCl_2.Closing2.Button_detection.Timer_LL.Counting -> (junction 70074)
            (junction 70074) -> (junction 70075) [order 2]
            (default) -> OpCl_doors.OpCl_2.Closing2.Button_detection.Timer_LL.Set
            OpCl_doors.OpCl_2.Closing2.Button_detection.Timer_LL.Set -> (junction 70076)
            (junction 70076) -> OpCl_doors.OpCl_2.Closing2.Button_detection.Timer_LL.Counting [order 1] : [ET_LL<PT_LL]
            (junction 70076) -> (junction 70075) [order 2]
          state BUTTON_DOWN
            state Button_DOWN_1
              en:
              BUTTON_DOWN(2)=true;
              BUT_TEMP=1;
              LPD1=true;
              PUSHED=true;
              UPDATE=false;
              IN_LL=false; ET_LL=0;
            state First_but_1
              en:
              BUT_1=BUT_TEMP;
              FIRST_BUT=false;
            state Button_DOWN_2
              en:
              BUTTON_DOWN(3)=true;
              BUT_TEMP=2;
              LPD2=true;
              PUSHED=true;
              UPDATE=false;
              IN_LL=false; ET_LL=0;
            state First_but_2
              en:
              BUT_1=BUT_TEMP;
              FIRST_BUT=false;
            state Button_DOWN_3
              en:
              BUTTON_DOWN(4)=true;
              BUT_TEMP=3;
              LPD3=true;
              PUSHED=true;
              UPDATE=false;
              IN_LL=false; ET_LL=0;
            state First_but_3
              en:
              BUT_1=BUT_TEMP;
              FIRST_BUT=false;
            (default) -> (junction 70089)
            (junction 70089) -> OpCl_doors.OpCl_2.Closing2.Button_detection.BUTTON_DOWN.Button_DOWN_1 [order 1] : [PD1]
            OpCl_doors.OpCl_2.Closing2.Button_detection.BUTTON_DOWN.Button_DOWN_1 -> (junction 70090)
            (junction 70090) -> OpCl_doors.OpCl_2.Closing2.Button_detection.BUTTON_DOWN.First_but_1 [order 1] : [FIRST_BUT && not(RPC1)]
            OpCl_doors.OpCl_2.Closing2.Button_detection.BUTTON_DOWN.First_but_1 -> (junction 70091)
            (junction 70089) -> (junction 70092) [order 2]
            (junction 70090) -> (junction 70093) [order 2]
            (junction 70091) -> (junction 70094)
            (junction 70093) -> (junction 70092)
            (junction 70094) -> (junction 70093)
            (junction 70092) -> (junction 70095)
            (junction 70095) -> OpCl_doors.OpCl_2.Closing2.Button_detection.BUTTON_DOWN.Button_DOWN_2 [order 1] : [PD2]
            OpCl_doors.OpCl_2.Closing2.Button_detection.BUTTON_DOWN.Button_DOWN_2 -> (junction 70096)
            (junction 70096) -> OpCl_doors.OpCl_2.Closing2.Button_detection.BUTTON_DOWN.First_but_2 [order 1] : [FIRST_BUT && not(RPC2)]
            OpCl_doors.OpCl_2.Closing2.Button_detection.BUTTON_DOWN.First_but_2 -> (junction 70097)
            (junction 70095) -> (junction 70098) [order 2]
            (junction 70096) -> (junction 70099) [order 2]
            (junction 70097) -> (junction 70100)
            (junction 70099) -> (junction 70098)
            (junction 70100) -> (junction 70099)
            (junction 70098) -> (junction 70101)
            (junction 70101) -> OpCl_doors.OpCl_2.Closing2.Button_detection.BUTTON_DOWN.Button_DOWN_3 [order 1] : [PD3]
            OpCl_doors.OpCl_2.Closing2.Button_detection.BUTTON_DOWN.Button_DOWN_3 -> (junction 70102)
            (junction 70102) -> OpCl_doors.OpCl_2.Closing2.Button_detection.BUTTON_DOWN.First_but_3 [order 1] : [FIRST_BUT && not(RPC3)]
            OpCl_doors.OpCl_2.Closing2.Button_detection.BUTTON_DOWN.First_but_3 -> (junction 70103)
            (junction 70101) -> (junction 70104) [order 2]
            (junction 70102) -> (junction 70105) [order 2]
            (junction 70103) -> (junction 70106)
            (junction 70105) -> (junction 70104)
            (junction 70106) -> (junction 70105)
          state BUTTON_CAR
            state Button_CAR_0
              en:
              BUTTON_CAR(1)=true;
              BUT_TEMP=0;
              LPC0=true;
              PUSHED=true;
              UPDATE=false;
              IN_LL=false; ET_LL=0;
            state First_but_0
              en:
              BUT_1=BUT_TEMP;
              FIRST_BUT=false;
            state Button_CAR_1
              en:
              BUTTON_CAR(2)=true;
              BUT_TEMP=1;
              LPC1=true;
              PUSHED=true;
              UPDATE=false;
              IN_LL=false; ET_LL=0;
            state First_but_1
              en:
              BUT_1=BUT_TEMP;
              FIRST_BUT=false;
            state Button_CAR_2
              en:
              BUTTON_CAR(3)=true;
              BUT_TEMP=2;
              LPC2=true;
              PUSHED=true;
              UPDATE=false;
              IN_LL=false; ET_LL=0;
            state First_but_2
              en:
              BUT_1=BUT_TEMP;
              FIRST_BUT=false;
            state Button_CAR_3
              en:
              BUTTON_CAR(4)=true;
              BUT_TEMP=3;
              LPC3=true;
              PUSHED=true;
              UPDATE=false;
              IN_LL=false; ET_LL=0;
            state First_but_3
              en:
              BUT_1=BUT_TEMP;
              FIRST_BUT=false;
            (default) -> (junction 70144)
            (junction 70144) -> OpCl_doors.OpCl_2.Closing2.Button_detection.BUTTON_CAR.Button_CAR_0 [order 1] : [P0]
            OpCl_doors.OpCl_2.Closing2.Button_detection.BUTTON_CAR.Button_CAR_0 -> (junction 70145)
            (junction 70145) -> OpCl_doors.OpCl_2.Closing2.Button_detection.BUTTON_CAR.First_but_0 [order 1] : [FIRST_BUT && not(RPC0)]
            OpCl_doors.OpCl_2.Closing2.Button_detection.BUTTON_CAR.First_but_0 -> (junction 70146)
            (junction 70144) -> (junction 70147) [order 2]
            (junction 70145) -> (junction 70148) [order 2]
            (junction 70146) -> (junction 70149)
            (junction 70148) -> (junction 70147)
            (junction 70149) -> (junction 70148)
            (junction 70147) -> (junction 70152)
            OpCl_doors.OpCl_2.Closing2.Button_detection.BUTTON_CAR.Button_CAR_1 -> (junction 70150)
            (junction 70150) -> OpCl_doors.OpCl_2.Closing2.Button_detection.BUTTON_CAR.First_but_1 [order 1] : [FIRST_BUT && not(RPC1)]
            OpCl_doors.OpCl_2.Closing2.Button_detection.BUTTON_CAR.First_but_1 -> (junction 70151)
            (junction 70150) -> (junction 70154) [order 2]
            (junction 70151) -> (junction 70155)
            (junction 70152) -> OpCl_doors.OpCl_2.Closing2.Button_detection.BUTTON_CAR.Button_CAR_1 [order 1] : [P1]
            (junction 70152) -> (junction 70153) [order 2]
            (junction 70154) -> (junction 70153)
            (junction 70155) -> (junction 70154)
            (junction 70153) -> (junction 70156)
            (junction 70156) -> OpCl_doors.OpCl_2.Closing2.Button_detection.BUTTON_CAR.Button_CAR_2 [order 1] : [P2]
            OpCl_doors.OpCl_2.Closing2.Button_detection.BUTTON_CAR.Button_CAR_2 -> (junction 70157)
            (junction 70157) -> OpCl_doors.OpCl_2.Closing2.Button_detection.BUTTON_CAR.First_but_2 [order 1] : [FIRST_BUT && not(RPC2)]
            OpCl_doors.OpCl_2.Closing2.Button_detection.BUTTON_CAR.First_but_2 -> (junction 70158)
            (junction 70156) -> (junction 70159) [order 2]
            (junction 70157) -> (junction 70160) [order 2]
            (junction 70158) -> (junction 70161)
            (junction 70160) -> (junction 70159)
            (junction 70161) -> (junction 70160)
            (junction 70159) -> (junction 70162)
            (junction 70162) -> OpCl_doors.OpCl_2.Closing2.Button_detection.BUTTON_CAR.Button_CAR_3 [order 1] : [P3]
            OpCl_doors.OpCl_2.Closing2.Button_detection.BUTTON_CAR.Button_CAR_3 -> (junction 70163)
            (junction 70163) -> OpCl_doors.OpCl_2.Closing2.Button_detection.BUTTON_CAR.First_but_3 [order 1] : [FIRST_BUT && not(RPC3)]
            OpCl_doors.OpCl_2.Closing2.Button_detection.BUTTON_CAR.First_but_3 -> (junction 70164)
            (junction 70162) -> (junction 70165) [order 2]
            (junction 70163) -> (junction 70166) [order 2]
            (junction 70164) -> (junction 70167)
            (junction 70166) -> (junction 70165)
            (junction 70167) -> (junction 70166)
          state BUTTON_UP
            state Button_UP_0
              en:
              BUTTON_UP(1)=true;
              BUT_TEMP=0;
              LPS0=true;
              PUSHED=true;
              UPDATE=false;
              IN_LL=false; ET_LL=0;
            state First_but_0
              en:
              BUT_1=BUT_TEMP;
              FIRST_BUT=false;
            state Button_UP_1
              en:
              BUTTON_UP(2)=true;
              BUT_TEMP=1;
              LPS1=true;
              PUSHED=true;
              UPDATE=false;
              IN_LL=false; ET_LL=0;
            state First_but_1
              en:
              BUT_1=BUT_TEMP;
              FIRST_BUT=false;
            state Button_UP_2
              en:
              BUTTON_UP(3)=true;
              BUT_TEMP=2;
              LPS2=true;
              PUSHED=true;
              UPDATE=false;
              IN_LL=false; ET_LL=0;
            state First_but_2
              en:
              BUT_1=BUT_TEMP;
              FIRST_BUT=false;
            (junction 70217) -> OpCl_doors.OpCl_2.Closing2.Button_detection.BUTTON_UP.Button_UP_0 [order 1] : [PS0]
            OpCl_doors.OpCl_2.Closing2.Button_detection.BUTTON_UP.Button_UP_0 -> (junction 70218)
            (junction 70218) -> OpCl_doors.OpCl_2.Closing2.Button_detection.BUTTON_UP.First_but_0 [order 1] : [FIRST_BUT && not(RPC0)]
            OpCl_doors.OpCl_2.Closing2.Button_detection.BUTTON_UP.First_but_0 -> (junction 70219)
            (default) -> (junction 70217)
            (junction 70217) -> (junction 70222) [order 2]
            (junction 70218) -> (junction 70220) [order 2]
            (junction 70219) -> (junction 70221)
            (junction 70221) -> (junction 70220)
            (junction 70220) -> (junction 70222)
            (junction 70222) -> (junction 70223)
            (junction 70223) -> OpCl_doors.OpCl_2.Closing2.Button_detection.BUTTON_UP.Button_UP_1 [order 1] : [PS1]
            OpCl_doors.OpCl_2.Closing2.Button_detection.BUTTON_UP.Button_UP_1 -> (junction 70224)
            (junction 70224) -> OpCl_doors.OpCl_2.Closing2.Button_detection.BUTTON_UP.First_but_1 [order 1] : [FIRST_BUT && not(RPC1)]
            OpCl_doors.OpCl_2.Closing2.Button_detection.BUTTON_UP.First_but_1 -> (junction 70225)
            (junction 70223) -> (junction 70226) [order 2]
            (junction 70224) -> (junction 70227) [order 2]
            (junction 70225) -> (junction 70228)
            (junction 70227) -> (junction 70226)
            (junction 70228) -> (junction 70227)
            (junction 70226) -> (junction 70230)
            OpCl_doors.OpCl_2.Closing2.Button_detection.BUTTON_UP.First_but_2 -> (junction 70229)
            (junction 70229) -> (junction 70234)
            (junction 70230) -> OpCl_doors.OpCl_2.Closing2.Button_detection.BUTTON_UP.Button_UP_2 [order 1] : [PS2]
            OpCl_doors.OpCl_2.Closing2.Button_detection.BUTTON_UP.Button_UP_2 -> (junction 70231)
            (junction 70231) -> OpCl_doors.OpCl_2.Closing2.Button_detection.BUTTON_UP.First_but_2 [order 1] : [FIRST_BUT && not(RPC2)]
            (junction 70230) -> (junction 70232) [order 2]
            (junction 70231) -> (junction 70233) [order 2]
            (junction 70233) -> (junction 70232)
            (junction 70234) -> (junction 70233)
          state Max_Min_assignment
            state Min_but
              en:
              BUTTON=MIN_BUT;
            state Max_but
              en:
              BUTTON=MAX_BUT;
            state First_but
              en:
              BUTTON=BUT_1;
            state Max_but1
              en:
              MAX_BUT=2;
            state Max_but2
              en:
              MAX_BUT=1;
            state Max_but3
              en:
              MAX_BUT=0;
            state Min_but1
              en:
              MIN_BUT=1;
            state Min_but2
              en:
              MIN_BUT=2;
            state Min_but3
              en:
              MIN_BUT=3;
            state MAX
              en:
              MAX_BUT=BUT_TEMP;
            state MIN
              en:
              MIN_BUT=BUT_TEMP;
            state Updating_button_0
              en:
              BUTTON=MAX_BUT;
            state Updating_button_1
              en:
              BUTTON=MIN_BUT;
            (junction 70272) -> OpCl_doors.OpCl_2.Closing2.Button_detection.Max_Min_assignment.Min_but [order 1] : [(MAX_BUT-FLOOR)>(FLOOR-MIN_BUT)]
            OpCl_doors.OpCl_2.Closing2.Button_detection.Max_Min_assignment.Min_but -> (junction 70273)
            (junction 70274) -> (junction 70272) [order 1] : [not(FLAG_STOP) && MOTION==2 && FLAG==3]
            (default) -> (junction 70274)
            (junction 70272) -> (junction 70275) [order 2]
            (junction 70273) -> (junction 70276)
            (junction 70274) -> (junction 70277) [order 2]
            (junction 70275) -> OpCl_doors.OpCl_2.Closing2.Button_detection.Max_Min_assignment.Max_but [order 1] : [(MAX_BUT-FLOOR)<(FLOOR-MIN_BUT)]
            OpCl_doors.OpCl_2.Closing2.Button_detection.Max_Min_assignment.Max_but -> (junction 70276)
            (junction 70275) -> OpCl_doors.OpCl_2.Closing2.Button_detection.Max_Min_assignment.First_but [order 2]
            (junction 70276) -> (junction 70279)
            OpCl_doors.OpCl_2.Closing2.Button_detection.Max_Min_assignment.First_but -> (junction 70278)
            (junction 70278) -> (junction 70277)
            (junction 70279) -> (junction 70278)
            (junction 70277) -> (junction 70280)
            (junction 70281) -> (junction 70282) [order 1] : [MOTION==0]
                | {MOTION=1;
                | UPDATE=true;}
            (junction 70282) -> OpCl_doors.OpCl_2.Closing2.Button_detection.Max_Min_assignment.Max_but1 [order 1] : [BUTTON_UP(2)]
            OpCl_doors.OpCl_2.Closing2.Button_detection.Max_Min_assignment.Max_but1 -> (junction 70283)
            (junction 70280) -> (junction 70281) [order 1] : [BUTTON==FLOOR && EXTEND]
                | {EXTEND=false;}
            (junction 70280) -> (junction 70294) [order 2]
            (junction 70281) -> (junction 70286) [order 2]
            (junction 70282) -> (junction 70284) [order 2]
            (junction 70283) -> (junction 70285)
            (junction 70284) -> OpCl_doors.OpCl_2.Closing2.Button_detection.Max_Min_assignment.Max_but2 [order 1] : [BUTTON_UP(1)]
            OpCl_doors.OpCl_2.Closing2.Button_detection.Max_Min_assignment.Max_but2 -> (junction 70285)
            (junction 70284) -> OpCl_doors.OpCl_2.Closing2.Button_detection.Max_Min_assignment.Max_but3 [order 2]
            (junction 70285) -> (junction 70288)
            OpCl_doors.OpCl_2.Closing2.Button_detection.Max_Min_assignment.Max_but3 -> (junction 70287)
            (junction 70287) -> (junction 70286)
            (junction 70288) -> (junction 70287)
            (junction 70286) -> (junction 70289)
            (junction 70289) -> (junction 70290) [order 1] : [MOTION==1]
                | {MOTION=0;
                | UPDATE=true;}
            (junction 70290) -> OpCl_doors.OpCl_2.Closing2.Button_detection.Max_Min_assignment.Min_but1 [order 1] : [BUTTON_DOWN(1)]
            OpCl_doors.OpCl_2.Closing2.Button_detection.Max_Min_assignment.Min_but1 -> (junction 70291)
            (junction 70289) -> (junction 70295) [order 2]
            (junction 70290) -> (junction 70292) [order 2]
            (junction 70291) -> (junction 70293)
            (junction 70292) -> OpCl_doors.OpCl_2.Closing2.Button_detection.Max_Min_assignment.Min_but2 [order 1] : [BUTTON_DOWN(2)]
            OpCl_doors.OpCl_2.Closing2.Button_detection.Max_Min_assignment.Min_but2 -> (junction 70293)
            (junction 70292) -> OpCl_doors.OpCl_2.Closing2.Button_detection.Max_Min_assignment.Min_but3 [order 2]
            (junction 70293) -> (junction 70297)
            OpCl_doors.OpCl_2.Closing2.Button_detection.Max_Min_assignment.Min_but3 -> (junction 70296)
            (junction 70295) -> (junction 70294)
            (junction 70296) -> (junction 70295)
            (junction 70297) -> (junction 70296)
            (junction 70294) -> (junction 70299)
            OpCl_doors.OpCl_2.Closing2.Button_detection.Max_Min_assignment.MAX -> (junction 70298)
            (junction 70299) -> (junction 70300) [order 1] : [PUSHED]
            (junction 70300) -> (junction 70301) [order 1] : [not(BUT_TEMP==FLOOR) || not(MOTION==2)]
            (junction 70301) -> OpCl_doors.OpCl_2.Closing2.Button_detection.Max_Min_assignment.MAX [order 1] : [MAX_BUT<BUT_TEMP && not(UPDATE)]
            (junction 70298) -> (junction 70303)
            (junction 70299) -> (junction 70313) [order 2]
            (junction 70300) -> (junction 70306) [order 2]
            (junction 70301) -> (junction 70302) [order 2]
            (junction 70303) -> (junction 70302)
            (junction 70302) -> (junction 70304)
            (junction 70304) -> OpCl_doors.OpCl_2.Closing2.Button_detection.Max_Min_assignment.MIN [order 1] : [MIN_BUT>BUT_TEMP && not(UPDATE)]
            OpCl_doors.OpCl_2.Closing2.Button_detection.Max_Min_assignment.MIN -> (junction 70305)
            (junction 70304) -> (junction 70307) [order 2]
            (junction 70305) -> (junction 70308)
            (junction 70307) -> (junction 70306)
            (junction 70308) -> (junction 70307)
            (junction 70306) -> (junction 70309)
            (junction 70309) -> OpCl_doors.OpCl_2.Closing2.Button_detection.Max_Min_assignment.Updating_button_0 [order 1] : [MOTION==0]
            OpCl_doors.OpCl_2.Closing2.Button_detection.Max_Min_assignment.Updating_button_0 -> (junction 70310)
            (junction 70309) -> (junction 70311) [order 2]
            (junction 70310) -> (junction 70312)
            (junction 70311) -> OpCl_doors.OpCl_2.Closing2.Button_detection.Max_Min_assignment.Updating_button_1 [order 1] : [MOTION==1]
            OpCl_doors.OpCl_2.Closing2.Button_detection.Max_Min_assignment.Updating_button_1 -> (junction 70312)
            (junction 70311) -> (junction 70314) [order 2]
            (junction 70312) -> (junction 70315)
            (junction 70314) -> (junction 70313)
            (junction 70315) -> (junction 70314)
          state GoTo_PositionControl
            en:
            BUTTON=BUT_TEMP;
            FLAG=2;
          state Emergency
            en:
            FLAG_EMG=true;
            FLAG=4;
          state Timer_EME
            state Set_tmr
              en:
              Q_EME=true;
            state Counting
              en:
              ET_EME= ET_EME + 1;
              Q_EME=false;
            state Set
              en:
              IN_EME=true;
              PT_EME=3;
            (junction 70405) -> OpCl_doors.OpCl_2.Closing2.Button_detection.Timer_EME.Set_tmr [order 1] : [ET_EME==PT_EME]
            OpCl_doors.OpCl_2.Closing2.Button_detection.Timer_EME.Set_tmr -> (junction 70406)
            OpCl_doors.OpCl_2.Closing2.Button_detection.Timer_EME.Counting -> (junction 70405)
            (junction 70405) -> (junction 70406) [order 2]
            (default) -> OpCl_doors.OpCl_2.Closing2.Button_detection.Timer_EME.Set
            OpCl_doors.OpCl_2.Closing2.Button_detection.Timer_EME.Set -> (junction 70407)
            (junction 70407) -> OpCl_doors.OpCl_2.Closing2.Button_detection.Timer_EME.Counting [order 1] : [ET_EME<PT_EME]
            (junction 70407) -> (junction 70406) [order 2]
          state Not_Emergency
            en:
            IN_EME=false;
            ET_EME=0;
          state SwitchingOFF_LEDs
            en:
            LPD3=false;
            LPD2=false;
            LPS2=false;
            LPD1=false;
            LPS1=false;
            LPS0=false;
          (default) -> (junction 70006)
          (junction 70006) -> (junction 70007) [order 1] : [FLAG==1 && not(PUSHED)]
              | {BUTTON=FLOOR;
              | BUT_TEMP=BUTTON;
              | BUT_1=FLOOR;}
          (junction 70007) -> OpCl_doors.OpCl_2.Closing2.Button_detection.Timer_LL [order 1] : [not(FLAG_STOP)]
          OpCl_doors.OpCl_2.Closing2.Button_detection.Save_energy -> (junction 70008)
          OpCl_doors.OpCl_2.Closing2.Button_detection.Timer_LL -> OpCl_doors.OpCl_2.Closing2.Button_detection.Save_energy
          (junction 70007) -> (junction 70010) [order 2]
          (junction 70006) -> (junction 70009) [order 2]
          (junction 70008) -> (junction 70011)
          (junction 70010) -> (junction 70009)
          (junction 70011) -> (junction 70010)
          (junction 70009) -> OpCl_doors.OpCl_2.Closing2.Button_detection.BUTTON_CAR
          OpCl_doors.OpCl_2.Closing2.Button_detection.BUTTON_UP -> OpCl_doors.OpCl_2.Closing2.Button_detection.BUTTON_DOWN
          OpCl_doors.OpCl_2.Closing2.Button_detection.BUTTON_DOWN -> OpCl_doors.OpCl_2.Closing2.Button_detection.Max_Min_assignment
          OpCl_doors.OpCl_2.Closing2.Button_detection.Max_Min_assignment -> (junction 70012)
          OpCl_doors.OpCl_2.Closing2.Button_detection.BUTTON_CAR -> OpCl_doors.OpCl_2.Closing2.Button_detection.BUTTON_UP
          (junction 70012) -> (junction 70014)
          (junction 70014) -> (junction 70013)
          (junction 70013) -> (junction 70016)
          OpCl_doors.OpCl_2.Closing2.Button_detection.GoTo_PositionControl -> (junction 70015)
          (junction 70016) -> (junction 70017) [order 1] : [FLAG==1]
          (junction 70017) -> OpCl_doors.OpCl_2.Closing2.Button_detection.GoTo_PositionControl [order 1] : [PUSHED]
          (junction 70015) -> (junction 70019)
          (junction 70016) -> (junction 70027) [order 2]
          (junction 70017) -> (junction 70018) [order 2]
          (junction 70019) -> (junction 70018)
          (junction 70018) -> (junction 70021)
          OpCl_doors.OpCl_2.Closing2.Button_detection.Emergency -> (junction 70020)
          (junction 70021) -> OpCl_doors.OpCl_2.Closing2.Button_detection.Timer_EME [order 1] : [STOP]
              | {IN_LL=false; ET_LL=0;FLAG=1;}
          OpCl_doors.OpCl_2.Closing2.Button_detection.Timer_EME -> (junction 70022)
          (junction 70022) -> OpCl_doors.OpCl_2.Closing2.Button_detection.Emergency [order 1] : [Q_EME]
          (junction 70020) -> (junction 70024)
          (junction 70021) -> OpCl_doors.OpCl_2.Closing2.Button_detection.Not_Emergency [order 2]
          (junction 70022) -> (junction 70023) [order 2]
          (junction 70024) -> (junction 70023)
          (junction 70023) -> (junction 70026)
          OpCl_doors.OpCl_2.Closing2.Button_detection.Not_Emergency -> (junction 70026)
          OpCl_doors.OpCl_2.Closing2.Button_detection.SwitchingOFF_LEDs -> (junction 70025)
          (junction 70026) -> OpCl_doors.OpCl_2.Closing2.Button_detection.SwitchingOFF_LEDs [order 1] : [FLAG_STOP && FLAG==2]
          (junction 70025) -> (junction 70029)
          (junction 70026) -> (junction 70028) [order 2]
          (junction 70028) -> (junction 70027)
          (junction 70029) -> (junction 70028)
        state Extending
          en:
          EXTEND=true;
        state Stop_Closing
          en:
          CP2=false;
          FLAG_OD=false;
          OBS=false;
          ET_cl=0;
          IN_cl=false;
        state GoTo_PositionControl
          en: FLAG=2;
        state GoTo_BUttonDetection
          en:
          MOTION=2;
          MAX_BUT=0;
          MIN_BUT=3;
          PUSHED=false;
          FIRST_BUT=true;
          FLAG=1;
          UPDATE=false;
        state Closing1
          en:CP2=true;
        state Stop_Closing1
          en:CP2=false;
        OpCl_doors.OpCl_2.Closing2.Reset -> OpCl_doors.OpCl_2.Closing2.Timer_close
        (default) -> (junction 69917)
        (junction 69917) -> OpCl_doors.OpCl_2.Closing2.Reset [order 1] : [not(FLAG==0) && not(FLAG==4)]
        OpCl_doors.OpCl_2.Closing2.Timer_close -> (junction 69918)
        (junction 69918) -> OpCl_doors.OpCl_2.Closing2.Closing [order 1] : [not(PC2)]
        OpCl_doors.OpCl_2.Closing2.Button_detection -> (junction 69919)
        OpCl_doors.OpCl_2.Closing2.Closing -> OpCl_doors.OpCl_2.Closing2.Button_detection
        (junction 69917) -> (junction 69927) [order 2]
        (junction 69918) -> (junction 69920) [order 2]
        (junction 69919) -> (junction 69925)
        (junction 69920) -> OpCl_doors.OpCl_2.Closing2.Extending [order 1] : [BUTTON==FLOOR]
        (junction 69920) -> (junction 69922) [order 2]
        OpCl_doors.OpCl_2.Closing2.Extending -> (junction 69921)
        (junction 69921) -> (junction 69922)
        (junction 69922) -> OpCl_doors.OpCl_2.Closing2.Stop_Closing
        OpCl_doors.OpCl_2.Closing2.Stop_Closing -> (junction 69923)
        (junction 69923) -> OpCl_doors.OpCl_2.Closing2.GoTo_PositionControl [order 2]
        (junction 69923) -> OpCl_doors.OpCl_2.Closing2.GoTo_BUttonDetection [order 1] : [not(BUTTON_CAR(1) || BUTTON_CAR(2) || BUTTON_CAR(3) || BUTTON_CAR(4) || BUTTON_UP(1) || BUTTON_UP(2) || BUTTON_UP(3) || BUTTON_DOWN(2) || BUTTON_DOWN(3) || BUTTON_DOWN(4))]
        OpCl_doors.OpCl_2.Closing2.GoTo_PositionControl -> (junction 69924)
        OpCl_doors.OpCl_2.Closing2.GoTo_BUttonDetection -> (junction 69924)
        (junction 69924) -> (junction 69925)
        (junction 69925) -> (junction 69926)
        (junction 69926) -> (junction 69928)
        (junction 69927) -> OpCl_doors.OpCl_2.Closing2.Closing1 [order 1] : [not(PC2)]
        OpCl_doors.OpCl_2.Closing2.Closing1 -> (junction 69928)
        (junction 69927) -> OpCl_doors.OpCl_2.Closing2.Stop_Closing1 [order 2]
        OpCl_doors.OpCl_2.Closing2.Stop_Closing1 -> (junction 69928)
      state StopClosing
        en: CP2=false;
        FLAG_OD=false;
      state Opening2
        state Opening
          en:AP2=Q_op;
        state People_IN
          state Check_People_IN
            en:
            COUNTER_IN=false;
          state People_KID_IN
            en:
            WEIGHT=WEIGHT+30;
            KIDS=KIDS+1;
          state People_WOMAN_IN
            en:
            WEIGHT=WEIGHT+55;
            WOMEN=WOMEN+1;
          state People_MAN_IN
            en:
            WEIGHT=WEIGHT+75;
            MEN=MEN+1;
          state People_FATGUY_IN
            en:
            WEIGHT=WEIGHT+100;
            FATGUYS=FATGUYS+1;
          state Re_Ready_IN
            en:
            COUNTER_IN=true;
          (default) -> (junction 89309)
          (junction 89309) -> OpCl_doors.OpCl_2.Opening2.People_IN.Check_People_IN [order 1] : [COUNTER_IN]
          OpCl_doors.OpCl_2.Opening2.People_IN.Check_People_IN -> (junction 89310)
          (junction 89310) -> OpCl_doors.OpCl_2.Opening2.People_IN.People_KID_IN [order 1] : [KID_IN]
          OpCl_doors.OpCl_2.Opening2.People_IN.People_KID_IN -> (junction 89311)
          (junction 89309) -> (junction 89318) [order 2]
          (junction 89310) -> (junction 89312) [order 2]
          (junction 89311) -> (junction 89313)
          (junction 89312) -> OpCl_doors.OpCl_2.Opening2.People_IN.People_WOMAN_IN [order 1] : [WOMAN_IN]
          OpCl_doors.OpCl_2.Opening2.People_IN.People_WOMAN_IN -> (junction 89313)
          (junction 89312) -> (junction 89314) [order 2]
          (junction 89313) -> (junction 89315)
          (junction 89314) -> OpCl_doors.OpCl_2.Opening2.People_IN.People_MAN_IN [order 1] : [MAN_IN]
          OpCl_doors.OpCl_2.Opening2.People_IN.People_MAN_IN -> (junction 89315)
          (junction 89314) -> (junction 89316) [order 2]
          (junction 89315) -> (junction 89317)
          (junction 89316) -> OpCl_doors.OpCl_2.Opening2.People_IN.People_FATGUY_IN [order 1] : [FATGUY_IN]
          OpCl_doors.OpCl_2.Opening2.People_IN.People_FATGUY_IN -> (junction 89317)
          (junction 89316) -> (junction 89319) [order 2]
          (junction 89317) -> (junction 89320)
          (junction 89319) -> (junction 89318)
          (junction 89320) -> (junction 89319)
          (junction 89318) -> (junction 89321)
          (junction 89321) -> OpCl_doors.OpCl_2.Opening2.People_IN.Re_Ready_IN [order 1] : [not(KID_IN|| WOMAN_IN || MAN_IN || FATGUY_IN)]
          (junction 89321) -> (junction 89322) [order 2]
          OpCl_doors.OpCl_2.Opening2.People_IN.Re_Ready_IN -> (junction 89323)
          (junction 89323) -> (junction 89322)
        state Timer_open
          state Set_tmr
            en: Q_op=true;
          state Set
            en:PT_op=2;
            IN_op=true;
          state Counting
            en:ET_op = ET_op + 1;
            Q_op=false;
          (junction 89358) -> OpCl_doors.OpCl_2.Opening2.Timer_open.Set_tmr [order 1] : [ET_op==PT_op]
          OpCl_doors.OpCl_2.Opening2.Timer_open.Set_tmr -> (junction 89359)
          (default) -> OpCl_doors.OpCl_2.Opening2.Timer_open.Set
          OpCl_doors.OpCl_2.Opening2.Timer_open.Counting -> (junction 89358)
          (junction 89358) -> (junction 89359) [order 2]
          OpCl_doors.OpCl_2.Opening2.Timer_open.Set -> (junction 89360)
          (junction 89360) -> OpCl_doors.OpCl_2.Opening2.Timer_open.Counting [order 1] : [ET_op<PT_op]
          (junction 89360) -> (junction 89359) [order 2]
        state Stop_Opening
          en:AP2=false;
          FLAG_OD=true;
          OBS=true;
          IN_op=false;
          ET_op=0;
        state People_OUT
          state Check_People_OUT
            en:
            COUNTER_OUT=false;
          state People_KID_OUT
            en:
            WEIGHT=WEIGHT-30;
            KIDS=KIDS-1;
          state People_WOMAN_OUT
            en:
            WEIGHT=WEIGHT-55;
            WOMEN=WOMEN-1;
          state People_MAN_OUT
            en:
            WEIGHT=WEIGHT-75;
            MEN=MEN-1;
          state People_FATGUY_OUT
            en:
            WEIGHT=WEIGHT-100;
            FATGUYS=FATGUYS-1;
          state Re_Ready_OUT
            en:
            COUNTER_OUT=true;
          (default) -> (junction 89374)
          (junction 89374) -> OpCl_doors.OpCl_2.Opening2.People_OUT.Check_People_OUT [order 1] : [COUNTER_OUT]
          OpCl_doors.OpCl_2.Opening2.People_OUT.Check_People_OUT -> (junction 89375)
          (junction 89375) -> OpCl_doors.OpCl_2.Opening2.People_OUT.People_KID_OUT [order 1] : [KID_OUT && KIDS>0 ]
          OpCl_doors.OpCl_2.Opening2.People_OUT.People_KID_OUT -> (junction 89376)
          (junction 89374) -> (junction 89383) [order 2]
          (junction 89375) -> (junction 89377) [order 2]
          (junction 89376) -> (junction 89378)
          (junction 89377) -> OpCl_doors.OpCl_2.Opening2.People_OUT.People_WOMAN_OUT [order 1] : [WOMAN_OUT && WOMEN>0]
          OpCl_doors.OpCl_2.Opening2.People_OUT.People_WOMAN_OUT -> (junction 89378)
          (junction 89378) -> (junction 89380)
          (junction 89377) -> (junction 89379) [order 2]
          (junction 89379) -> OpCl_doors.OpCl_2.Opening2.People_OUT.People_MAN_OUT [order 1] : [MAN_OUT && MEN>0]
          OpCl_doors.OpCl_2.Opening2.People_OUT.People_MAN_OUT -> (junction 89380)
          (junction 89379) -> (junction 89381) [order 2]
          (junction 89380) -> (junction 89382)
          (junction 89381) -> OpCl_doors.OpCl_2.Opening2.People_OUT.People_FATGUY_OUT [order 1] : [FATGUY_OUT && FATGUYS>0]
          OpCl_doors.OpCl_2.Opening2.People_OUT.People_FATGUY_OUT -> (junction 89382)
          (junction 89381) -> (junction 89384) [order 2]
          (junction 89382) -> (junction 89385)
          (junction 89384) -> (junction 89383)
          (junction 89385) -> (junction 89384)
          (junction 89383) -> (junction 89386)
          (junction 89386) -> OpCl_doors.OpCl_2.Opening2.People_OUT.Re_Ready_OUT [order 1] : [not(KID_OUT || WOMAN_OUT || MAN_OUT || FATGUY_OUT)]
          (junction 89386) -> (junction 89387) [order 2]
          OpCl_doors.OpCl_2.Opening2.People_OUT.Re_Ready_OUT -> (junction 89388)
          (junction 89388) -> (junction 89387)
        state Button_detection
          state Save_energy
            en:
            LL=not(Q_LL);
          state Timer_LL
            state Set_tmr
              en:
              Q_LL=true;
            state Counting
              en:
              ET_LL= ET_LL + 1;
              Q_LL=false;
            state Set
              en:
              IN_LL=true;
              PT_LL=10;
            (junction 89491) -> OpCl_doors.OpCl_2.Opening2.Button_detection.Timer_LL.Set_tmr [order 1] : [ET_LL==PT_LL]
            OpCl_doors.OpCl_2.Opening2.Button_detection.Timer_LL.Set_tmr -> (junction 89492)
            OpCl_doors.OpCl_2.Opening2.Button_detection.Timer_LL.Counting -> (junction 89491)
            (junction 89491) -> (junction 89492) [order 2]
            (default) -> OpCl_doors.OpCl_2.Opening2.Button_detection.Timer_LL.Set
            OpCl_doors.OpCl_2.Opening2.Button_detection.Timer_LL.Set -> (junction 89493)
            (junction 89493) -> OpCl_doors.OpCl_2.Opening2.Button_detection.Timer_LL.Counting [order 1] : [ET_LL<PT_LL]
            (junction 89493) -> (junction 89492) [order 2]
          state BUTTON_DOWN
            state Button_DOWN_1
              en:
              BUTTON_DOWN(2)=true;
              BUT_TEMP=1;
              LPD1=true;
              PUSHED=true;
              UPDATE=false;
              IN_LL=false; ET_LL=0;
            state First_but_1
              en:
              BUT_1=BUT_TEMP;
              FIRST_BUT=false;
            state Button_DOWN_2
              en:
              BUTTON_DOWN(3)=true;
              BUT_TEMP=2;
              LPD2=true;
              PUSHED=true;
              UPDATE=false;
              IN_LL=false; ET_LL=0;
            state First_but_2
              en:
              BUT_1=BUT_TEMP;
              FIRST_BUT=false;
            state Button_DOWN_3
              en:
              BUTTON_DOWN(4)=true;
              BUT_TEMP=3;
              LPD3=true;
              PUSHED=true;
              UPDATE=false;
              IN_LL=false; ET_LL=0;
            state First_but_3
              en:
              BUT_1=BUT_TEMP;
              FIRST_BUT=false;
            (default) -> (junction 89506)
            (junction 89506) -> OpCl_doors.OpCl_2.Opening2.Button_detection.BUTTON_DOWN.Button_DOWN_1 [order 1] : [PD1]
            OpCl_doors.OpCl_2.Opening2.Button_detection.BUTTON_DOWN.Button_DOWN_1 -> (junction 89507)
            (junction 89507) -> OpCl_doors.OpCl_2.Opening2.Button_detection.BUTTON_DOWN.First_but_1 [order 1] : [FIRST_BUT && not(RPC1)]
            OpCl_doors.OpCl_2.Opening2.Button_detection.BUTTON_DOWN.First_but_1 -> (junction 89508)
            (junction 89506) -> (junction 89509) [order 2]
            (junction 89507) -> (junction 89510) [order 2]
            (junction 89508) -> (junction 89511)
            (junction 89510) -> (junction 89509)
            (junction 89511) -> (junction 89510)
            (junction 89509) -> (junction 89512)
            (junction 89512) -> OpCl_doors.OpCl_2.Opening2.Button_detection.BUTTON_DOWN.Button_DOWN_2 [order 1] : [PD2]
            OpCl_doors.OpCl_2.Opening2.Button_detection.BUTTON_DOWN.Button_DOWN_2 -> (junction 89513)
            (junction 89513) -> OpCl_doors.OpCl_2.Opening2.Button_detection.BUTTON_DOWN.First_but_2 [order 1] : [FIRST_BUT && not(RPC2)]
            OpCl_doors.OpCl_2.Opening2.Button_detection.BUTTON_DOWN.First_but_2 -> (junction 89514)
            (junction 89512) -> (junction 89515) [order 2]
            (junction 89513) -> (junction 89516) [order 2]
            (junction 89514) -> (junction 89517)
            (junction 89516) -> (junction 89515)
            (junction 89517) -> (junction 89516)
            (junction 89515) -> (junction 89518)
            (junction 89518) -> OpCl_doors.OpCl_2.Opening2.Button_detection.BUTTON_DOWN.Button_DOWN_3 [order 1] : [PD3]
            OpCl_doors.OpCl_2.Opening2.Button_detection.BUTTON_DOWN.Button_DOWN_3 -> (junction 89519)
            (junction 89519) -> OpCl_doors.OpCl_2.Opening2.Button_detection.BUTTON_DOWN.First_but_3 [order 1] : [FIRST_BUT && not(RPC3)]
            OpCl_doors.OpCl_2.Opening2.Button_detection.BUTTON_DOWN.First_but_3 -> (junction 89520)
            (junction 89518) -> (junction 89521) [order 2]
            (junction 89519) -> (junction 89522) [order 2]
            (junction 89520) -> (junction 89523)
            (junction 89522) -> (junction 89521)
            (junction 89523) -> (junction 89522)
          state BUTTON_CAR
            state Button_CAR_0
              en:
              BUTTON_CAR(1)=true;
              BUT_TEMP=0;
              LPC0=true;
              PUSHED=true;
              UPDATE=false;
              IN_LL=false; ET_LL=0;
            state First_but_0
              en:
              BUT_1=BUT_TEMP;
              FIRST_BUT=false;
            state Button_CAR_1
              en:
              BUTTON_CAR(2)=true;
              BUT_TEMP=1;
              LPC1=true;
              PUSHED=true;
              UPDATE=false;
              IN_LL=false; ET_LL=0;
            state First_but_1
              en:
              BUT_1=BUT_TEMP;
              FIRST_BUT=false;
            state Button_CAR_2
              en:
              BUTTON_CAR(3)=true;
              BUT_TEMP=2;
              LPC2=true;
              PUSHED=true;
              UPDATE=false;
              IN_LL=false; ET_LL=0;
            state First_but_2
              en:
              BUT_1=BUT_TEMP;
              FIRST_BUT=false;
            state Button_CAR_3
              en:
              BUTTON_CAR(4)=true;
              BUT_TEMP=3;
              LPC3=true;
              PUSHED=true;
              UPDATE=false;
              IN_LL=false; ET_LL=0;
            state First_but_3
              en:
              BUT_1=BUT_TEMP;
              FIRST_BUT=false;
            (default) -> (junction 89561)
            (junction 89561) -> OpCl_doors.OpCl_2.Opening2.Button_detection.BUTTON_CAR.Button_CAR_0 [order 1] : [P0]
            OpCl_doors.OpCl_2.Opening2.Button_detection.BUTTON_CAR.Button_CAR_0 -> (junction 89562)
            (junction 89562) -> OpCl_doors.OpCl_2.Opening2.Button_detection.BUTTON_CAR.First_but_0 [order 1] : [FIRST_BUT && not(RPC0)]
            OpCl_doors.OpCl_2.Opening2.Button_detection.BUTTON_CAR.First_but_0 -> (junction 89563)
            (junction 89561) -> (junction 89564) [order 2]
            (junction 89562) -> (junction 89565) [order 2]
            (junction 89563) -> (junction 89566)
            (junction 89565) -> (junction 89564)
            (junction 89566) -> (junction 89565)
            (junction 89564) -> (junction 89569)
            OpCl_doors.OpCl_2.Opening2.Button_detection.BUTTON_CAR.Button_CAR_1 -> (junction 89567)
            (junction 89567) -> OpCl_doors.OpCl_2.Opening2.Button_detection.BUTTON_CAR.First_but_1 [order 1] : [FIRST_BUT && not(RPC1)]
            OpCl_doors.OpCl_2.Opening2.Button_detection.BUTTON_CAR.First_but_1 -> (junction 89568)
            (junction 89567) -> (junction 89571) [order 2]
            (junction 89568) -> (junction 89572)
            (junction 89569) -> OpCl_doors.OpCl_2.Opening2.Button_detection.BUTTON_CAR.Button_CAR_1 [order 1] : [P1]
            (junction 89569) -> (junction 89570) [order 2]
            (junction 89571) -> (junction 89570)
            (junction 89572) -> (junction 89571)
            (junction 89570) -> (junction 89573)
            (junction 89573) -> OpCl_doors.OpCl_2.Opening2.Button_detection.BUTTON_CAR.Button_CAR_2 [order 1] : [P2]
            OpCl_doors.OpCl_2.Opening2.Button_detection.BUTTON_CAR.Button_CAR_2 -> (junction 89574)
            (junction 89574) -> OpCl_doors.OpCl_2.Opening2.Button_detection.BUTTON_CAR.First_but_2 [order 1] : [FIRST_BUT && not(RPC2)]
            OpCl_doors.OpCl_2.Opening2.Button_detection.BUTTON_CAR.First_but_2 -> (junction 89575)
            (junction 89573) -> (junction 89576) [order 2]
            (junction 89574) -> (junction 89577) [order 2]
            (junction 89575) -> (junction 89578)
            (junction 89577) -> (junction 89576)
            (junction 89578) -> (junction 89577)
            (junction 89576) -> (junction 89579)
            (junction 89579) -> OpCl_doors.OpCl_2.Opening2.Button_detection.BUTTON_CAR.Button_CAR_3 [order 1] : [P3]
            OpCl_doors.OpCl_2.Opening2.Button_detection.BUTTON_CAR.Button_CAR_3 -> (junction 89580)
            (junction 89580) -> OpCl_doors.OpCl_2.Opening2.Button_detection.BUTTON_CAR.First_but_3 [order 1] : [FIRST_BUT && not(RPC3)]
            OpCl_doors.OpCl_2.Opening2.Button_detection.BUTTON_CAR.First_but_3 -> (junction 89581)
            (junction 89579) -> (junction 89582) [order 2]
            (junction 89580) -> (junction 89583) [order 2]
            (junction 89581) -> (junction 89584)
            (junction 89583) -> (junction 89582)
            (junction 89584) -> (junction 89583)
          state BUTTON_UP
            state Button_UP_0
              en:
              BUTTON_UP(1)=true;
              BUT_TEMP=0;
              LPS0=true;
              PUSHED=true;
              UPDATE=false;
              IN_LL=false; ET_LL=0;
            state First_but_0
              en:
              BUT_1=BUT_TEMP;
              FIRST_BUT=false;
            state Button_UP_1
              en:
              BUTTON_UP(2)=true;
              BUT_TEMP=1;
              LPS1=true;
              PUSHED=true;
              UPDATE=false;
              IN_LL=false; ET_LL=0;
            state First_but_1
              en:
              BUT_1=BUT_TEMP;
              FIRST_BUT=false;
            state Button_UP_2
              en:
              BUTTON_UP(3)=true;
              BUT_TEMP=2;
              LPS2=true;
              PUSHED=true;
              UPDATE=false;
              IN_LL=false; ET_LL=0;
            state First_but_2
              en:
              BUT_1=BUT_TEMP;
              FIRST_BUT=false;
            (junction 89634) -> OpCl_doors.OpCl_2.Opening2.Button_detection.BUTTON_UP.Button_UP_0 [order 1] : [PS0]
            OpCl_doors.OpCl_2.Opening2.Button_detection.BUTTON_UP.Button_UP_0 -> (junction 89635)
            (junction 89635) -> OpCl_doors.OpCl_2.Opening2.Button_detection.BUTTON_UP.First_but_0 [order 1] : [FIRST_BUT && not(RPC0)]
            OpCl_doors.OpCl_2.Opening2.Button_detection.BUTTON_UP.First_but_0 -> (junction 89636)
            (default) -> (junction 89634)
            (junction 89634) -> (junction 89639) [order 2]
            (junction 89635) -> (junction 89637) [order 2]
            (junction 89636) -> (junction 89638)
            (junction 89638) -> (junction 89637)
            (junction 89637) -> (junction 89639)
            (junction 89639) -> (junction 89640)
            (junction 89640) -> OpCl_doors.OpCl_2.Opening2.Button_detection.BUTTON_UP.Button_UP_1 [order 1] : [PS1]
            OpCl_doors.OpCl_2.Opening2.Button_detection.BUTTON_UP.Button_UP_1 -> (junction 89641)
            (junction 89641) -> OpCl_doors.OpCl_2.Opening2.Button_detection.BUTTON_UP.First_but_1 [order 1] : [FIRST_BUT && not(RPC1)]
            OpCl_doors.OpCl_2.Opening2.Button_detection.BUTTON_UP.First_but_1 -> (junction 89642)
            (junction 89640) -> (junction 89643) [order 2]
            (junction 89641) -> (junction 89644) [order 2]
            (junction 89642) -> (junction 89645)
            (junction 89644) -> (junction 89643)
            (junction 89645) -> (junction 89644)
            (junction 89643) -> (junction 89647)
            OpCl_doors.OpCl_2.Opening2.Button_detection.BUTTON_UP.First_but_2 -> (junction 89646)
            (junction 89646) -> (junction 89651)
            (junction 89647) -> OpCl_doors.OpCl_2.Opening2.Button_detection.BUTTON_UP.Button_UP_2 [order 1] : [PS2]
            OpCl_doors.OpCl_2.Opening2.Button_detection.BUTTON_UP.Button_UP_2 -> (junction 89648)
            (junction 89648) -> OpCl_doors.OpCl_2.Opening2.Button_detection.BUTTON_UP.First_but_2 [order 1] : [FIRST_BUT && not(RPC2)]
            (junction 89647) -> (junction 89649) [order 2]
            (junction 89648) -> (junction 89650) [order 2]
